simulink model "Noa_Nofusion_backup"  (R2020b)
settings: Solver=FixedStepDiscrete  StartTime=0.0  StopTime=Inf  FixedStep=0.02  RelTol=1e-3
PostLoadFcn:
  | if any(exist('dsrtsu_mdlpostloadfcn', 'file') ~= 0), dsrtsu_mdlpostloadfcn('Execute', bdroot); end
InitFcn:
  | , if any(exist('rtifpga_mdlclblib', 'file') ~= 0), rtifpga_mdlclblib('Init', bdroot); end,
  | , if any(exist('dsmpb_private', 'file') ~= 0), dsmpb_private('dsmpb_mdlclblib', 'Init', bdroot); end,
undefined symbols (not defined in the file): ACC_TimeGap_DecSetSwt, ACC_TimeGap_IncSetSwt, AccelPedalPosn, AccelPedalPosnVldty, AccelPedlPosnDiagc, AccPedalOverride, ACU_ShiftInProgress, ADAS_Posn_CurLane, AESSwtReq, ALC_SwtReq, BrkPedalSts, CC_ACC_CANCEL_OFFSwt, CC_ACC_CRUISE_OFFSwt, CC_ACC_DecSetSpd_SetSwt, CC_ACC_IncSetSpd_ResuSwt, CC_ACCSwtErr, CharSpd_ms, CSA_NODE, CURRENT_GEAR, CurrentGearValid, DiscIntNeverNeededParam, DrvDoorSts, DrvSBR, DrvTrqReqOvld, ECMACCInterface, ECMRespACC, ELKSwtReq, EngLimpHomeSts, EngSpd, EngState, EngState_PHEV, EngTrqMaxActSpd, EngTrqMinAct, EPS_DrvInpTrqVal_HighReslolution, EPS_FailSts, EPS_LKATorqOvrlDlvd, EPS_LKATorqOvrlDlvdVld, EPS_LKATrqOvlDlvdSts, EPS_SteerMod, EPS_TrqSnsrSts, EQ4_APPINFO, EQ4_LA_ELEM, EQ4_LA_HDR, EQ4_LAP_ELEM, EQ4_LAP_HDR, EQ4_LH_ELEM, EQ4_LH_HDR, EQ4_LRE_ELEM, EQ4_LRE_HDR, ESS_PedSwtReq, ESS_VehSwtReq, FFogLmpSts_F_Pbox, FLWheelDriveDirection, FLWheelSpd, FrntWiprSwtSts, FrntWshrSwtSts, FRWheelDriveDirection, FRWheelSpd, HazardLmpSwtSts, HCU_AccelPedalPosn_Diag ... (+152)
libraries: simulink x117, dsmpblib x30
(part 1 of 11)
PreSaveFcn:
  | , if any(exist('dsmpb_private', 'file') ~= 0), dsmpb_private('dsmpb_mdlclblib', 'PreSave', bdroot); end,
CloseFcn:
  | , if any(exist('dsmpb_private', 'file') ~= 0), dsmpb_private('dsmpb_mdlclblib', 'Close', bdroot); end,
settings Model: DataDictionary=HWA_DDs.sldd  RTICANMMDATA=struct('GeneralSetupData',struct('modelroot','D:\ADAS_Store\Project\adas_project','generalsettings',struct('filesettings',struct('destfolder',struct('Name','RTICANMM_FILES','Check',1),'buildfolder',struct('Name','.','Check',1),'AbsDestfolder',struct('Name','D:\ADAS_Store\Project\adas_project\RTICANMM_FILES'),'AbsBuildfolder',struct('Name','D:\ADAS_Store\Project\adas_project'))),'options',struct('addpaths',1,'rmpaths',1,'addtrcexclusion',false,'cannavigator',struct('checkmonitoring',0),'show_usrtrc',0,'use_usrtrc',0),'advanced',struct('options',ones(1,100)),'MPSetup',{{}},'RTI',struct('Type','DSRT','Ver','4.4','Date','02-Nov-2020'),'modelname','Noa_Nofusion','block','Noa_Nofusion'))  DSRTSU_INTERNAL_RTIFPGA=170  DSMPB_ID_DATA={'105434',struct('BlockId','e4345bf9-5197-4b1e-bd44-61eb3726c26b','SignalIds',{{'26e03e37-8c74-4456-a1ca-96577a784511','08c7dde7-a79a-486f-a58d-e9b634b8613f','1f5a9323-8244-4deb-bd12-eda6c6bbb4b7','bc7a83a0-3632-4f82-8cb2-387644efddca','463d03f2-aaf4-4ca5-834a-63a22e0dbd24','ff01abf3-987a-416d-8eb9-6d8f794c440d','a2437182-dc0c-46c3-ac4d-08683593369c','67741761-aed5-4514-b3bb-eb9079150845','4cc3f4fa-5aab-4adc-a725-9d1cb733df4e','fdc02adf-bcbe-4b15-b2ae-adf627f92255','a032f0fc-e186-436f-afc3-d181db7ca0f9','1cb07c07-79d8-437d-98ef-a715fe9ea012','b05a5e47-f50f-478a-a637-5469c5388606','f41b7890-420b-4a6b-8009-0b5652f97978','d622c0c0-f466-4673-93ce-b079da25035e','71aba0d3-083a-41fc-8fbc-153153d0300d','adb1eff1-8bdf-4208-b3d8-aca34dde9050','a3da7591-6b53-4fcf-b698-0e5273c81e81','a998d2a0-6de8-4bd6-b5ac-dc2d5f8f6b74','5e2ab582-2ba3-4786-882d-7e45b79ee759','0c4ff3f6-444f-4552-8419-c424fcf95c3f','d1700e2b-2e44-4df0-90ee-8a8e8a240ee1','4011d0ea-7b24-40b1-b899-1ec42639ad6f','c062954e-3331-410a-8824-613eb22a1fc5','16bc174b-a18e-43b6-985b-a64a73e0a52f','cfaca706-1dd7-407d-a107-3e9967b0bc1a','a67fec9e-f77d-4ccf-86bb-46fdce40b352','150cab41-1ab5-4854-ac2c-feddb3f5cac9','58e8d9c3-1336-475b-a3f9-01b1e0314959','42e83e1a-7335-4d70-b47f-232895adc5a7','e777976c-f6c2-4f04-a8b7-d94d8ccf44be','91bdfc1f-659c-4474-96fa-ea1cd21ec91f','20a78a99-30de-4c30-936b-ec269208d6d7','8b4dfdb2-a3a4-415e-85d2-0017a012fe9c','bfe8ea3b-4428-481b-a2cf-ef431c2d4e88','a4dae870-9959-4a91-8cf5-9cb1a03dd0d0','bd415c22-eb37-430d-9fba-56a2024eab30','32c5bc48-1ef1-4e48-92fe-e0b8bf641969','b8824d59-4ff1-44f9-9d43-98ccd1ef7818','2b530dc6-df14-4df3-a10d-b6a7a38ee3a9','47fc8431-8e5b-40fe-9bef-bd4f615a5465','85a00529-8abf-480a-b50f-da5245136546','75671914-23b0-4c0a-acae-2b7d58b763e3','69d46c2d-3b92-4b7a-8592-6c17caf294ed','18268954-c92f-4566-9cfe-583b74be0081','2fbcbfd7-1e0f-462c-b4b5-155ea0e0a8e3','851a228b-4320-48ca-8076-5eaf54d60810','99d04a46-e5a2-472b-a0f2-fbb65c8254da','e47a005c-a981-49a8-95c2-c7622c1b877c','b894dada-0a4e-47c5-adc8-0014d2607e23','0ac0dd78-1a61-4124-a84e-c4d508ff7f6c','dfe863a0-dbf9-4271-9fdd-b9d8c3f7cc2c','3669fba7-b792-4083-b91c-6483b65952fa'}}),'105435',struct('BlockId','d40121bf-53fc-4e4c-bf6b-9841f4415676','SignalIds',{{'cc5a11f6-e480-49b4-bcb9-da409be93ad0','e485a1c5-525b-420d-b245-0bdec7efe4d1','7063e335-e5a3-4215-a027-5b046a440513','370c96c2-c68f-4ad4-b008-588ba83deb3f','29c9a21f-53c2-4740-9418-e0028da600c3','d2ec761d-b188-4679-8bab-e24c9a56caed','fb0e0b0d-7187-4054-93dc-12a477d09059','0587543f-c20a-4b2c-a9d7-421455e1177c','c6236804-cf03-4372-979f-22949d9ffe47','dde724cd-4d84-43d6-9098-33f65af196ff','456acbbc-8be7-49b5-a0d4-6e3481273074','0fbd5400-87a8-4635-a5b6-02b9f8aa8a25','70bf8bc3-6666-425f-b514-d1e4a0a78933','6f4a0559-72ca-4952-81c7-e8c921498f82','ba6e8235-f42a-4def-b53d-6a69067deba9','3d993282-3ed7-4dce-a9ee-645c134cd44b','0cc06f80-c240-43a4-9b8f-4f6b9595cd8a','053b5169-944f-400b-bfa1-e4821136ec08','57d9f0be-2eb9-404e-becf-fcabc8470df5','b6e2025d-94a1-4f04-bfad-ebc0c3406e95','d9141aee-70c6-4284-a507-75d7f7a00e1e','6081e494-0e08-4c0c-ab2a-c6f970f11c8d','9fb5f869-4a24-4422-be73-f89fea30026b','a31ae767-f7c2-4d08-b138-f5b138cd782c','8978b272-f1d1-4dda-9a18-2e5bf203213e','fcb4403e-c5c0-4e63-a493-c28f06f4e989','e95a9918-a651-41d3-ae0a-66028e446d9c','83432099-6253-4fca-888f-af4b2b218d19','42653c93-2326-41ae-baca-2973fac6a4de','8836ad72-f3ce-4aae-b8a2-47c801e52c02','b0c13cb1-1574-4c16-b62e-ae7ad4d8b61f','283ef39f-4105-462c-ab0a-cf33dde3f661','3b3621be-a1a5-446e-a438-ee9142b86be2','43a4c43b-4ff0-45de-8a39-183cfd89222b','f08aa7ec-d521-4475-a3ac-08ba9d0ef18c','b2db309d-0a89-48d7-8b02-3a67f6913b10','2755c593-1eee-4c99-b46a-f03229636a7f','e2fd6a35-f7f1-4726-95a6-4e08663ad70a','abca7ea8-e11e-4d27-af8b-de618eedc876','b658c1af-14c2-430b-a331-ada145c0fea0','f98fe55d-f2a9-4261-90b9-8c4000dd9d04','688c6ece-80a2-46b2-af42-176bf1f9fd39','e9d10bd0-a7c8-403c-8590-31b64efec433','304f842a-dd0a-46f4-9fe1-0b3ef7066bf8','7a2840a9-195b-4485-bc10-ebd18e7a7110','6d0cfa48-0ecb-4659-a5ec-3cf69aa05638','00a37eaf-aba1-44b0-861e-c63e2cf71b26','f01dd479-691e-4b24-b10f-fb2a411ef3f9','bd845b67-c975-41c8-99fa-8d1e7106f6bc','4f7fdd21-b181-405f-9b00-d96648cb766b','f3389090-f0b9-457c-85ae-bcafb5f9c756','4657600f-e2ac-49c3-8fcf-c6d5ad3031eb','1a617fb4-0046-4c94-8581-01a2871ceae9','010eda22-fdee-4a99-b239-11724803971c','a9e798ca-198f-4a95-aa52-b8bf9c198389','f780cb99-b180-495d-b16b-9a32fb4fc008','946e88ec-8a2f-445c-887d-8b232953bb76','0cf59188-d479-4f11-b384-9398ad11b0b9','b429280c-67f5-4e1b-9e7e-07e7eafab7b3','c68f2587-46cf-4460-91be-325a9f6f0058','31916026-ab7c-4d26-b8d9-7c0947af4bb6','4056ca2d-ee20-4a0e-b887-5f2d42dcd476','0722f49f-64d1-446e-bcc5-e32cefc2cd07','9aa8ee7a-4d05-4864-bf05-1bde538fb5ef','91f59306-c587-4cfa-8cca-f2fa2bb27640','3ce34415-7470-4bbf-b6a0-34b9c9680686','2521a64c-fa73-4f46-8f58-43774ca93d19','22f357ae-cedf-4c71-a114-455f7eeeb852','f33afee2-1018-43a1-b2f2-b8249068a706','a3099f95-10d5-484f-9bcc-6a12ed409148','1c44e4b8-1a98-47ad-9d1c-ea3a539f74b4','cbbdc108-b603-452b-a824-5e42f89503e4','fff7e395-1071-48e3-909e-1e745a3936a4','a01a96d1-a628-4ae1-bc97-285a27885103','98d1c28e-f030-4320-a1d9-6263669e6f95','d3664eaa-a3c1-4179-98f6-7c6d4c30bddd','813f9209-a7ab-41be-85e3-3427ba85c434','18fe41b5-a649-45f3-bbfc-b0dbc7cb99ae','72475f52-be41-464a-8f0e-e9a62708a4e8','dad4bb40-ec9c-4aaf-9fc2-0712ec0f2241','4ab7dcd5-e52e-4fcb-ac29-82510b47df2f','7a00036e-29f5-4968-8d52-2a0ca2bfb714','4a83fb4c-b02f-4893-a8ea-dc9fd0347245','1294e5c8-6cb6-4f97-af30-ed027a407515','c1586ad9-805f-4123-af29-7bd37ac08373','fd82f8eb-65d1-4726-94d6-6ed5227b2f44','71f76165-f05e-444f-b18f-bd431ae3420a','9ca8daaa-938c-4c2c-b40f-9abb9fa373dc','a275610e-c197-4c68-93df-f8647aab9abe','4e816bd2-5b5b-4838-8c15-47e708c09655','107a9ec9-74cc-42d8-9479-17c41f92d23a','3f69883d-5772-4566-8b65-fe213494fc07','1acadf61-6fdd-4c01-b3d0-7293d5cf0b9d','fb5d8406-dead-4a01-914e-d88103fdc350','5b74708a-44f5-4ce1-bf13-9f0606d646a8','849bf2a4-7bc4-4e70-8423-14ca390664cd','a62a9267-333d-4d26-851d-bc457f3b81f8','1e129e98-37c9-4fc9-818c-296032360fc6','a4650b49-c80e-4b85-9076-c990629bae0d','c0ee05c1-f0cb-4541-aaf7-6d6b08f9a5cd','e2d169c4-0d8b-4400-a269-692e3f91bbe6','492a74b3-4d11-4662-8c3b-fde7cb230339','819494d0-34e1-4282-a222-1b52ba27ccab','5a638eb9-ccad-4d4a-9718-d37c62ee852b','c803a847-ecfa-4cce-960c-e106f0c4ea6f','e886af01-08d7-4704-a3ee-2d930691e91b','96070339-ef94-4b80-bb03-79310102b68a','b439ed2b-cdd1-4b08-990d-2a205f128d33','032805cc-419f-403c-9f6a-0eca3a183b61','88916648-e457-4bfb-9eef-162e217cdd8d','0c495062-db58-4a97-9a48-9d285bff8853','a627fe6a-96e3-480d-a583-a27d3bea5d25','799f7d78-721d-4d18-9b5b-df25b89a1a24','0365b900-2f19-45b4-8da9-34546021be40','0fff78c4-c430-446f-9f7e-7cf1c2560c13','bb3dcfc4-42bd-4e8e-9b87-b5baa2fa9966','f58a7d4f-359d-4f5a-a673-ecae1cec1cff','29bfd316-2c17-4da6-ac7c-92a41147bdbd','10fce9c2-b244-4020-bbae-d37dc28ebbc1','02e3f3c5-b52c-40f5-bf8b-7c169b6a050b','d1869188-5151-488a-974b-611ef2b3e735','3feb2bce-f837-4d53-afcb-2f51abb1249b','17ce8e05-201a-4ce1-90ef-a5d5fde36f30','cd40ee62-3fd3-4019-9f81-335d24b7e533','77bdded1-20d9-44f7-bebc-305e6f8a7542','7fb625b1-1694-40d9-8650-06db9adf04b9','0e5ce812-dc7b-4bcd-b991-c5485d68b836','fee2eb9c-0478-4758-b416-366bfd0a0b08','36b53c99-ed23-40ea-b736-d6080d358e52','7a9ac993-3f27-46ec-a0be-48db83299b68','720de45d-04c1-463b-9803-ef9b2b0640e6','48dd3c23-1521-4de4-8c14-bbfe09d8cdd3','0cf887f5-6df1-4e9b-89ca-8de50e244c96','d3e92529-0445-49a6-ae88-b8db65620ada','00961a9b-8e43-41d7-9361-0f7c9a191df1','176a2a26-953b-451b-bee7-639fa5dcf115','05743b62-48ad-4976-855d-4efd760ab5ae','5c8a3068-7b46-4863-96ad-cb43b0bebbf8','7e50c02a-d315-4f98-9ab4-c963b22f5fd1','decd5ca8-ac57-4887-88b5-f572b41815e6','7df3046e-b8b8-48de-bf08-08b163efbe98','068e11f8-fc7c-478e-a264-2eba7fdaf707','75e971b6-9816-4b6d-894c-7f0a5e23aad8','1245d556-b9a4-4269-8015-ee1cf4c77d66','e7a9388a-c9d2-45d1-b0c1-14f92e703417','e3451999-4f34-4207-a06a-a1a02f4ebc46','095f9967-1705-4584-a3c0-0a7a58bb2f86','a03cfd89-db34-40c1-9760-adbbbd92ecf4','2f200d12-fadd-4c60-b392-739715aba906','dab68d27-ce17-4104-94fb-d9520fd1074c','19930cd6-7971-4ea0-b243-faaedad380b0','81ee13d2-2426-454b-896a-4e968cc2b063','2182b590-601e-4655-89eb-6887a470e591','1cbdb8e1-bb61-4c18-a563-629debd208b5','94606876-5750-4d63-9bf3-4013ab9917c7','3146120c-38a4-4420-939c-eda38ea68cb3','cdb35835-5fbf-4349-a86b-fb87a21169b8','d21c81c0-6dba-44be-b882-848afe41626b','1201d19a-6fe5-41bd-ae3a-bd6a13dff8b8','91a5b005-6117-4516-a073-8851c35bf8a8','06b71312-9340-475e-b4be-cd3240c14140','23eb5363-a588-4710-961d-f99ccdee6ff8','a9d3dd51-03fa-4728-ae9b-f934500f1552','7be770a8-e416-43fc-a2aa-3a7b7d47063f','b1cd6e8c-2dc7-441e-8774-2b064ee9434b','77f2dd4e-5295-4873-839c-2804f01636cc','ccb8cb5c-6d49-4f47-9128-08c71a8596c2','68b38d10-57c2-46cd-a9a3-39ab701353d7','6d2417b2-923b-4307-8e62-1a997f2a7e41','057f6026-574a-4c10-b798-8674bc70fe4a','4ad31521-ed04-4046-afa9-acec64e978f6','53b9bb73-2211-4cd3-9be8-cc07ee60870f','fb200ae3-4897-4a2e-aa8f-753c4cb12daf','f1dd6b03-29f1-4510-9072-d50a6fa7b5cc','b4da77c0-2abc-4e81-9be0-4fa0d3784d94','ece98af3-fed9-4289-8066-50dff056db58','021a28ab-d2b0-4e56-906a-085143f1e294','9ad79b1c-39a9-41eb-926a-7326bbcf277b','6607879f-b8a8-470e-baed-66e05d35583a','fa2f7a6f-8388-4a48-ad80-d1f0da9fad28','d494d8ac-ce0c-4623-bb94-131d0977ba58','0cccf5e1-0fdc-4153-9508-5cf92d457e81','7407a7e1-6edd-4d87-b55c-fcdd84c2983f','9a18cd5b-06a3-4c13-9bcf-7adb69bb1915','453e0b8f-8cc9-4c76-9632-9981e365a1fe','a1003730-fcc8-4975-85c0-d51f67bec0e9','d1e041e3-d630-4ed2-a4a1-3340570a9861','24f6b2e2-26d0-40b7-91d3-4d06786d847c','44224ffc-9120-4fa4-823b-43d88ecfae98','ed8d8980-8de8-47c8-8352-9a2594ec7e8d','4594a42e-3277-4356-960d-db7f54018581','b7933dfc-e99b-4671-ac5b-0b539745cf2e','debde9d5-90eb-48ab-b125-b2c5ad0b1089','b175ca9d-34d9-40b6-8ff5-919b9d14b24d','5177fe90-62fd-4f07-9408-1db74678403b','439b298e-d093-4fc9-bc29-09baf018ca0a','fec7866a-292c-4ddb-8b2e-f6973b69ef06','a11ede85-44f0-4b05-85ec-a5bd55f71b4f','a0cc3722-caa3-40e0-a9fb-a0bf80e1730e','63ffd194-2be4-4603-904d-59907a931c27','d969c761-cb58-4b59-b72d-b3777adbeb2e','fd61477a-d646-4fa6-aa14-daa7a0500d24','e597bce3-f71b-4756-9897-14f096504c8b','c8c59d5b-acf9-4b59-b898-f2cf904d292e','0161e9c2-c134-4633-8f84-d49d04144a87','8b756ca8-0e95-427b-8560-8d1f79dc86da','9fcac863-048e-40ae-9155-08ed5010dc46','be979dbb-77e6-409c-8d46-a282d6d7b717','9e1fe4da-8bf4-415b-bf54-a00fc9538685','6ed6f9c2-07e6-42c9-9d33-83aecc381688','17e8478b-6bb3-4189-9dd7-157df52c13c6','f1bdca73-12af-435d-b22d-32002e65f1ee','929a8c7c-97c0-44c7-8c79-fd6a80dca632','413238d4-e9da-4389-8fa2-056224cdc256','56cabf32-638a-46a9-abe3-0f9647e0cd12','3ce98a47-237f-42c0-ade4-ef06ae0e8951','eebaa124-7f65-4430-9871-33a15f887caa','d4e60423-8c8f-45b6-b121-b99db76df8fb','cc5a559f-a448-4899-906f-5dc9e1af9340','e974851a-54fb-475f-ad1c-f92776865502','ca0cf790-84fd-46f7-a553-c999687b713a','8ca16ee8-27ae-46d4-8d1b-6484f0ba2e1c','759c7fa4-ecac-423f-8cc7-22d8663b1b7d','a32945fc-842a-404d-b759-2c4082d0afb1','a3e8dd22-699f-447d-8e26-c3e63e8cdf8d','c7e4f5ce-5fc0-4b2d-8595-25b0d014f116','2afbdbf5-e43f-49a0-92c2-dbf86f141ee2','a67f7783-5f44-41b0-b0e5-610b7cd4cf93','28fa3106-f248-4371-864f-c995c3c6a1d8','c92b734f-8e2d-4b7e-9242-c73c51499704','41b74adc-ad96-4fa8-a326-67da154d2e5a','9c6b6b81-d000-40da-a81f-97b7769edeb7','3fcb895b-97d5-422c-8812-44e5092a1c13','425b0fc0-c480-477f-8574-0f601cf6a832','ac0d790f-a75e-4b8c-8140-f1a1077511fb','907c9527-8a89-4c72-9ec5-032b21f4476e','01f35774-1138-4815-9226-b549d6d07300','9c2c0849-8eb5-489f-9256-4c61f1511d6c','691b024e-ea18-47b8-8c91-4d9a84de3391','8ce8ee90-d8ac-4999-be4a-3cc9b1a1ddd5','330b6441-7005-41d8-8d7e-c2fe0fa98f1e','097751a8-dab4-48de-be29-ce5c72bfa38f','ea9e5656-c12c-4b65-b5b0-27911e1a9074','d894742d-141c-4ca1-a31d-14590af5cb88','18db3a2f-1f99-45ff-a28c-9d4de5ca09f2','bd93bda1-440c-42c1-a94b-31318096355d','c9010752-1ccc-4f48-9d88-00800dca04af','3dbf7699-72c3-4cd8-a1ed-344c2b193fab','6e11cc67-229d-49fe-9524-842e8beb6dbd','5c6911d4-ec52-457f-abc4-7531c8e96b32','3642b32f-b4ad-4eda-87e5-e57e269a0737','3ce9a289-c5d9-4dc9-a836-09cb77dba024','6b1c0f1c-5802-4a48-928a-7d14e45f2140','21de2f49-14de-4bcd-bfd3-ac7f7ebcc380','3585a489-3f47-4b9b-99f8-630657ca6b61','d2933102-4f42-4f86-bd5e-5f2f55fca8a9','c441195f-73a4-4dde-bfdb-1e99f2d402de','2bd35363-f924-48df-9bf7-0ff957eaa548','8fdd4ce3-583b-4977-bfd4-267de9e56221','da41d479-773c-4ae6-b31c-6f2c310b8697','5197f87c-2bad-4e3e-b8eb-1dee0cc507a1','0b6746dd-4b7d-4483-b390-2596ea9c94f6','d3aaca7a-e726-45c6-a876-1d36405328e8','e4c351a4-0d06-418c-b290-86601264d4e9','98a41ba7-8f43-4ee2-b203-f62db5551338','319d5c62-7a79-4fd4-8ace-256e219e7927','a704a474-bc59-4be4-9c29-cb9a85f8ed60','0b2a3c92-dc27-4033-9d0f-76ea27442d02','437b8219-2177-46a7-8e27-d74badf66ad7','bdfda334-42ae-4382-a6d1-596cda2fae0f','3ce29b3e-42e1-40a8-a4a5-c1706b66ef27','c9c7185d-6b37-4c0a-8b35-64238a1ec5cd','76a3b79d-a942-4f96-8d54-397cb6d54134','69332480-af1c-4431-8c89-956bc5b9ada2','b90b99c2-80b5-41f4-b872-e8d40f6b986f','11904823-be19-4a56-b728-0959cc99c2dd','007e0102-eb7a-460e-bd55-efc54a9d09c9','2dff0e5b-5a66-4099-a59f-03486706e809','ab438635-fcd0-49c1-b5d7-3a38a6dd5d6c','a8ce4e02-4111-4410-bb37-aeb5015d0f28','4612e75f-7972-4b2a-b0d7-cc8e529f0a42','0946edce-7d00-4b41-9bc2-d0551a007d3b','838dbe22-0353-4e26-a393-dea5335713dc','eddf385a-eb65-4c84-8f9f-cfc6e10ae678','83670045-0068-4c9d-9d44-ca98496249c4','6ad6d159-db55-406e-b158-d7decc68f78d','22db6a37-3350-4ca4-a97b-07980acf5a21','512fea98-8afc-49e2-a79d-9818b29f3894','692e8e3f-1d4a-4455-a7c7-e545a1ba0b9a','251c595e-841d-428b-ba31-7c6b9e852587','764d5c32-5c5e-4761-9071-007a4bc162d6','1f53d17f-2a1c-4bee-8a7d-dc4d7147df35','e51b0e47-7399-47cd-b026-f67ad625f364','2861a8b7-810c-4ce0-a0c0-b0502751c142','1c517d95-89a7-4442-9e57-b93e98d12f2c','8a9ac90b-68ea-474f-aee3-1e5008fd098d','d0c1cfbf-c955-475e-bed2-714d1c907249','74d6c0be-dcbb-4737-a584-266dd9978f33','b654b6a2-8011-4d6c-8572-18d135e251ed','91b173c3-804f-4276-9f17-2d6da234f79e','69a1db0f-61e5-461f-bba8-b382b8817f9d','c451186f-65aa-46d6-9d99-cec024e2d63d','79c91a5e-f416-40d0-976b-045ec1d133d9','c2a92a7d-2bd8-4d7d-addc-c31bbe7b2e06','add2c099-0616-4f5e-a06e-a2a69bd83097','a85fa2d7-93f4-4009-901e-c7991975856a','9b79f2a7-b3dd-46bc-b8c5-92d7ffe34ab8','e61b549a-71d7-4ce5-b867-e409b4815d6a','6e0eb462-856a-420e-806e-2aefdaa6f9e9','59708c7f-a4f8-439d-bbd5-ef006d9d94e5','53a689a5-895b-4661-a768-18b97131f9b5','d63e55a5-23fa-4d36-848f-48eb2a0b39ef','01c1f276-f558-49cc-8256-1ae84a7c9a8f','fb911f03-0812-43ff-be03-aef72409e834','53ca8056-b924-4d6c-9003-fd141a5a0e09','f502775a-ea5f-4fc8-8f49-0d44588d6923','fd9a4963-42bf-454b-9105-f84f7d212dbf','8d2ad19f-788c-4d41-86a3-6f5092c3659a','c0569295-9bbc-41d6-9c4d-9217cc984067','08af115d-a552-4fc9-a13e-9bbb52271bbc','d5b4cbab-f87c-47a9-91f6-fea75233e2d1','17487a72-6383-4c65-8972-21fa963fbec0','10d55baa-318c-42d3-a564-e728fe9d2880','ed40f1ae-203a-4951-a78c-f63f8a19583b','8a0734ac-6aaf-4db4-9ab3-f1d7de829468','9be2a3ee-f28d-470e-9b68-7e167ab84867','c4ffb54d-ed0f-457f-851c-5f221df9afce','3486935b-dd1c-489b-bbd3-73e6da203050','405ea1cd-827d-4205-9f8b-6d069b3358ef','65b16e84-ab72-4179-aea2-fbfb6032235d','77256c6e-1bae-412b-8946-ade2dfcd8b2b','a8569a15-8d34-4499-a902-3b93742385d6','29f4f5f1-a2f0-4d17-a8d2-e5bd679a6191','32be050f-77e3-418b-8fc0-01d52c0f81b1','5299eb59-fdbd-40fb-a2de-98847db328fd','c2270d11-788e-4144-9bfe-f73fc87d227c','f4e19d23-2bd5-45f8-a648-acae3bbe24a8','ce4d68ff-941f-4558-9f31-d5b994b2288c','32445c74-1dc3-44dc-80ff-d2d906b6c70b','3e688b65-7195-46bc-af07-3a64420f53b6','e63a5e33-f993-4f75-82f4-28d25c86114b','a10fa038-6d5a-4d31-a99e-1ababa1005ec','b4a17c3f-7bec-4608-93f6-1a3701a46531','afca4047-6d67-42e4-a93d-21200c4aa8dc','14830bc3-064a-4486-b298-24319e1b19e4','7227227c-9520-4bb3-ac59-8e658092cb02','9b8b4492-a383-43ed-b6e9-5de3f8b2d5e0','cf459a79-3a7d-4d6e-a941-a4e0299de77e','5f828eec-cf46-46a6-9017-894a0d3527a0','db4f20b4-b889-454d-a614-d932461c028b','e7defd96-dc06-4b27-b5c8-0cca9e849e3f','5c1cacc8-6dc4-4385-939f-f931d9898e3b','f2f4044e-2c02-422e-a838-b2c8cb3726e1','93e34572-36f4-418e-8e83-15f4a80aff5d','2300ce0d-9c26-4d74-a513-69e4f5a4cd51','e13b9b7d-ff74-4822-8ac5-33be9ab3de9b','30c78f0a-e43b-4ca4-a84d-6db014e323ae','872e4fe2-02f8-40bd-bd6b-e2ac1f3bf7aa','e8115592-43a3-46d2-b96e-27f73a6523bf','43175569-a76a-4ac4-a1cd-f6b9a9e75f9e','42b25d4f-daa9-4294-a50b-017c03fda841','8ed3fbe7-accd-404d-8895-c45f61cd0cec','f68c054c-bb02-42c8-a359-37c399b89720','87971450-497c-412c-bf6f-8b77d211ec78','87db29d9-3059-41f1-917b-22bf2a621b77','3c6509ea-4a7f-4b60-9eb8-89f60a25992b','94f6b9b8-e704-4ddc-a645-cb1ae885c6ef','0948a254-3f43-4540-8864-8dd051921852','f9fd1072-82c8-4ba9-a8e9-745ab72c9d76','ed2d49be-d164-48bd-84f7-69a0a497bce8','545e9a80-fa65-4761-beeb-1097ab7b8a0e','bc2f1593-2577-4309-b83e-d05fee864886','2fc0fbbd-b198-43f4-9475-a901d5a10df6','9448c0e2-d8b4-4b68-97ba-7566a4a369b5','2474c5c6-41bc-41d2-aad8-465a46f2299c','524230cd-ca9f-4540-a678-50e3a691675a','35027490-03c2-4e93-9285-d408e3c85e64','5025e79e-722c-4608-b43d-2901a71948d0','b0480f38-c56a-4d59-ac9f-ee8a3a1c57c0','1f90e26d-0793-4665-a0de-7a98851a40b7','3a1ed6d3-3604-4d4a-9fc8-f094d7b31959','75b3eeb1-22b6-4b60-b443-5fe2744cd2df','44c2b35c-5090-48f9-bcaa-8050a1aa8fce','2b74c30b-cae2-4bcb-9a6a-98002332f100','547621c3-903e-48fd-a997-48378e062f62','fa9d664d-76fc-4f25-9f93-7dbf800054b0','93723c2f-03eb-4897-a44c-6d71daaf449d','ee3dc453-bece-4de9-b121-84375ee9e7da','fd4d0393-b60d-442f-bbe2-0f7f41acbc47','276fdf0e-63b2-4701-87b9-5ac3544636da','0c15af05-1b72-45e1-bfa5-9f7fe0e5fbd2','b9b2465d-5d27-4f91-913a-bee1615fd701','8df75123-e18f-480f-9d47-c0cb24e5dee7','77900ef1-cac5-4a18-96ec-1e3969270f79','024ddc86-7b33-4e29-8e87-0331e33b85b9','eb91361b-cc72-4174-95d9-9350d6ba38bb','1aecc688-47a9-4060-b8d2-3c94e7dbf89b','38ea6185-827f-4fa3-b4c7-83b5994143c2','f0517fc1-3e6c-4f3a-815c-dc1aa8a54192','d6c1d36c-d6e8-4461-9d0e-865617157fc6','9002abc6-6fca-4f66-94a4-ecabafa6ad9b','a1b25a5d-d9e8-40ed-8aa2-53d788e19b80','640fb393-c1b7-41f4-865d-09736c3d80ec','2fe3441a-504b-4e78-9135-3c2fda2e2fd5','4a6cd03b-2dd2-40fe-9040-0f0de504e462','3129f584-06a9-491b-9699-308a3f45a965','872ad8ed-c974-4495-ac7e-2a5b2ba741d9','20d2934c-1584-4be4-9879-ffb0fbe83803','e605361b-6cc4-4f26-b248-1db43a5454aa','fef12649-2b55-476d-8333-d82f5b554505','9cd47144-1de7-4899-a9e9-97d887f8d469','1313e814-b848-4453-a121-d9f1a42e2af0','0857829a-9dee-4edf-96c2-6b6bb5e76e34','8b45f3ee-ca72-4f72-8edc-f82059d0336c','9282acc7-127b-493c-98bb-8d88a1013977','945d9a30-6007-43d8-8e08-e078ab5d64de','a3fa0d28-3aff-4251-ac7d-7c64d54c7559','6c2ebdd8-afeb-4ea2-aa66-f7da39f68241','872b1e63-7e3b-41af-a38a-3982289009bc','3b7278aa-5f7b-44c5-90df-cd506fa3f5fc','6e30a5ac-5d6b-42ae-87b0-afd320eeaeab','0a6da5ec-bd82-46a3-9eda-f18aebda6601','78517c35-3059-4ba9-971a-45ff1196bccb','f79b8480-ffc7-4d29-b810-bcec72590bdf','093d2339-c1b2-4c9e-b437-c400b15b4f4d','eebb9dfb-1c5e-49fa-896b-e5fba41c1b70','1fa49630-a0be-4d70-9bd4-d900160c129b','4df3d1eb-f3f3-4780-af48-82697afcfa11','177dcbd7-e619-4a30-9b13-afd4e8f4c2fa','5e930fd7-66a6-427e-91c8-105a61db1d96','645914d5-a509-4680-81ab-634d41dde3c6','a2e12e22-9ba2-40f4-a1f7-4665d552aba3','debf0d17-6936-48bd-9d3f-d919662e03ec','8c5a8513-e35a-49cc-9947-5a1ff1e951e9','1c774eaa-e026-492d-a7e1-166124c32074','f5ca4b0d-deb3-41cc-accb-9a1ee16adc68','c96534b0-3f4a-44cc-bae1-4a1e802d61bb','038c2574-5fac-4a3d-8ba3-010f8d57dd9c','e91099a2-4c9b-48a5-8441-7df00938d62f','328eaf6e-c2ad-4ce7-b942-5ee57fc74870','f0947079-c6b9-4f20-aa56-bf3017b22ab4','b7e450fd-76ee-4981-a166-6259c51a50b4','ff84976c-67b2-4e04-9479-0083e5aafcc6','a8b0654d-e895-43fc-a680-2d8c731d149e','181a7022-ad56-43df-9b78-b64aa88713be','fc1bdf5a-b163-4486-9b91-03b0ab9c4023','ac8d2dd7-6153-4b07-87f6-4c3afed3e8e5','aa078f9b-9919-40e0-916e-c537e33a147b','b1873af7-21b3-4d95-b938-327be1c75b3b','ce70938a-10a0-41ad-943e-05e03baff434','f98eaa4c-5183-43f0-b63c-14b71790f611','b28686c5-02f6-454d-b057-1d675bdb81dc','e501155d-e3db-4bdb-95fd-d9622615055f','997faa46-b2de-4896-8e20-c2d4b8c1359c','fa78a12b-5d1e-4dee-bb17-1834b3c8f455','f72b09e6-6ccf-4d0f-a41f-ed679523f25e','d0021c27-2b6b-4827-b51d-7dae07425cd3','0ca30b9a-ece4-4689-a30b-96b0d9ce0167','96cbe83f-e04a-49c0-bff2-9623662c59f8','7433a08b-ca56-4233-a44a-5fa434f0b0b6','cda9548b-ecad-400f-ad22-55d4d1a3034c','492e642e-f9a2-48ce-b4df-bedb1adba8f9','d0eed24d-8ae1-4b25-8b6c-dcd5cf2c5ada','a4b28015-5085-4a81-8cc7-6144387ae4df','c38c694e-03d4-41bd-a9bc-a768a6c88d12','6e4029f7-4175-4233-98dd-fb097fa48970','89aca7a1-29c5-4954-9aa0-a670cc06e716','31944a79-b71b-462b-a6a1-9700eaa7b622','b2edd40b-d14e-4ddc-9b97-fd5aba5bd231','6bac8ba3-2f15-4911-8c3d-ba8376aa477c','f637f810-4adf-411b-aac1-4200ea0fe85b','f7602eb6-4760-46ec-b2c2-317c91bcc786','9dbcd6b5-bdf9-4599-a1b6-2e160dfa39ce','d2d6003e-c548-4ca8-a3d3-dccf5b598c1c','41daca08-c47d-4b8d-b345-a256e3c9be05','1f0b2279-0d5e-4443-8e9a-bc2fb4132a04','ec850a1f-c1ef-4b95-be8c-0e656818072e','7c975cac-4371-44ea-8053-0fd7bbd0c0fe','c243ed10-3bcf-49a3-8d67-2c142b11082f','5c646964-a426-41a3-9ce9-c215cb224a48','2d2fbae8-b398-4b6b-abfb-92d613fe18c4','a1435485-97e9-4877-b32d-304fb55e593b','94e98a66-7a74-4ced-8799-14727150fceb','b28c0b82-b79d-4816-8282-c74a0faeb3ec','f88e3e0d-a5c5-499c-a41f-2d1f925246f2','153af746-85d0-482a-b09b-76e153e776ce','5b91d707-8005-4e2e-8c86-118f89bcd2cd','36a32770-064e-4ecf-b363-c380a63312e5','11e4ff97-3c1d-4677-b9f5-389b298367da','c8ca6a3b-6d79-45da-a732-19ebe7540d7a','2f3df6e4-689d-42df-9d33-abf61f398c17','aeac4155-96c1-42fb-bc91-dc2c71c84578','2f8672f1-293a-40fa-bc35-85313a8da8bb','22dae23c-75cc-4ecf-a50f-aac362affbc7','c61b4382-846b-4a4f-a77b-e32e101667d1','611c4c25-17ff-4a12-8ca5-5537c3f7172c','750fa776-02e6-43a3-9fc1-ad672310e662','ab405c98-81db-45e4-80f0-a92434826387','e614b9e2-9e69-48a3-922a-c5f7752510a7','fdfda15b-f0cd-4cbe-b404-792dc2b0bed3','98f0ebe3-81d2-4b78-9d87-74cf0084b6e9','2e44af90-6a82-44c6-aa8c-2bc22f022714','61fc0436-4c82-430a-9722-a740790c8c14','370892f2-7549-465d-998b-a2ce99efc57d','f1e6264e-da30-4cee-a00b-a5f83ac3e8e5','066d2082-dfc3-44ed-b147-fc69905c3c5f','532d65e0-6f07-4992-92df-b9a9a018e250','1d3c285d-4537-4ac5-a3e4-edbdc625ce6c','08111893-6837-40ed-8b40-f1ef204607d4','74c0ee99-93c3-48fa-919c-c3a9f11ba173','de9b029b-0dc5-4540-b986-f626842d6427','a8cdf389-57bd-49d2-a453-f9dc5d1e984a','dcad49b6-d164-4790-ab28-5cdbfa2bb824','4a544db2-2a77-4ff9-a04e-7108a1e0bee7','181caa71-36e7-49f3-bcb7-56d2cc5f1505','b61f2922-2c0f-4312-b4de-12f0c4c94267','488d3233-de64-4ced-92c0-f77b27a88278','b7a15496-bf48-4f94-b60d-d9beda9e5839','2bf98379-1a31-45b3-9a7e-b57fea12a2cd','c1fedad6-6467-4ffe-a048-214609bc09dc','82097f1a-66e7-4b40-b629-4c21dbeb3a8f','d4f185be-a131-408b-8361-9f9cff72d4cd','3110e54e-5590-4dea-83ac-73b3a08d0550','4890fde5-f133-4e4e-a86b-6e5b7d44a980','08f31489-3abe-4937-92ab-b313d1c8c012','c145d1cb-19fb-4ff0-a8e3-e01cc887bb19','9e22bb75-4dd1-455d-b275-77b1b32c4e6a','34864cab-f8f4-4255-a26a-ac1bb9d8945b','281987eb-75a2-414e-b987-1b9bfddecadf','182a94a1-b8d9-4d51-8323-75170b59bdb1','9bb3641f-7eaa-4291-88ff-e1e3387bd97a','a6c1bac4-6fa8-47cc-b077-c21d524b49ee','a7fbbc63-2495-49fb-b72f-95b96116a0bf','1224b643-5da6-42ae-bbc1-55fe86bd58c6','c47c2fa8-0fea-41f9-92d6-66869a1b68d0','7096924f-0dfd-43cd-811a-980c70179f14','82158df1-abba-45cc-b849-4b2a0579f252','f300e8f1-a702-44b8-9dee-2712171c3a4c','3203aaad-c207-4d6b-9bd1-5bc965399be9','58ff5499-9242-40b5-bdad-d0e3fc167ceb','d443acd8-a96c-4fb6-ac01-451f0684ac31','f679937c-2064-4dec-8be6-f76b0e38263e','fd084c7d-eb86-4368-8e97-e1c7add861d4','95323bef-95d2-4714-9850-37a27cec1544','b6d7a45e-92d1-40fd-99f6-765a36cbb47a','f57bb77f-370c-4610-8cb1-4ddf2d9b3f74','1e8d914c-245c-4031-a0c8-f41917af18dc','85eda06c-09a8-438c-84a4-adebf7f77bc9','7521dc8e-0f81-4410-8079-d12e65789e30','e5049629-49f9-42d1-9f17-438bbc9e756c','fd432edd-8ed8-45dd-8c0f-7ca243305c4c','3ee7e66c-50bb-4821-a59e-049d581d339f','7522269c-3161-41bf-86d0-d958e12ac46a','cb333743-0f34-4d2e-8ba0-9d785247386d','398c7213-7966-4355-9cc9-7df5df0a75cf','d6994e42-c094-4dbe-8462-0da62a6a2e14','ae025030-5835-479e-a891-de27c637d219','61c95da0-80a2-46bd-97e1-9e6ad24f03ee','f2a29bec-b092-4ee4-9fe6-fce02dce5ed4','e269417a-cb48-427b-832e-5a14eb272aa0','6959e6bb-5c9f-4b9b-bd79-e26a56b76732','7ac261e6-cb91-4dae-90ac-c3704f71ddd1','6dd6c97e-d3ba-4bcb-b804-a10871f2db2e','21e7cfda-c211-4274-88b8-f3f4cba0bd14','a6123d7e-4449-4f75-bf5e-d90c2380af46','a18abd56-433c-454b-90b4-c4778833004f','efd2caff-f245-4b85-9947-5cac4b28862f','91ab604c-c6bc-47f5-981b-c349fa72b926','7765fab9-c597-4b3f-8c58-0b616b9aca52','32eb21df-1468-4f8f-b80b-0132e79946c4','23461d37-abcb-4de2-93b6-2c5b9b0285c5','2f82fe29-cbeb-4541-889b-8ca434b5dcdc','3aa5c75c-7fb8-475d-9ad8-74a6ef58f588','15702135-bba1-410e-9bd8-8a29575c5c9c','35d807ff-7560-4d31-aaf3-ad2e714f519e','f48fcd4f-b01a-4034-bca8-7150444f550f','36733f44-25e4-4e8f-9e06-a4eb4e366c81','9eb18c40-97e9-4722-8ada-89233fc24c6e','944672f7-8fdf-4c70-a203-1adb1ce43a88','46b707f3-17e0-4422-bdd0-c1515277267a','238ce7a8-54b8-4006-be0f-3c4ba43785ff','b4d4ebce-d852-41fa-b6b4-2d67323f73ba','480a575a-bb13-409f-8c82-179fad07672f','19788773-3210-44b5-bd38-6bbec63a8a33','2e9dd13d-b0c8-4b4d-b372-2c82b162cb3f','e675fb90-8b87-4e7c-85cd-6f23e0c28968','d593f8d6-dec2-4410-9bda-9b883f31f0ca','301d845b-2e55-4696-a79f-a33255234f38','15f9d93e-2322-4578-b26b-89a96a6236ed','e9aa8cfc-a767-4491-899f-76f9d70f9d6d','f6b3c952-7eae-40af-b06e-142c6ce86f9f','e59c1f00-1b72-4967-9c9e-0acfcff55407','3e5f55da-2125-4567-a48f-328cef8365e1','9e510b27-5ca4-450c-8f27-456defee6958','e1a18f76-2953-40fc-a9b5-cdc760845927','c032c242-3216-416f-98aa-6193bbda84bf','a5351ad5-64be-40f8-9ec4-28c814d50f85','1ed74a08-4f3b-40c4-bd2c-10e1ee884d6a','4bb619bf-cfb1-43c1-b123-98b1567fdeb1','4b011f18-a11e-4ac7-a14e-a7dedc986832','85c53582-83bb-43b3-a48a-5a6f6c021d88','e0841b18-6478-4e07-9646-269550b47938','1781b9e6-7833-4278-8d2c-4f594bde1b7e','e26c4ef4-feeb-48f4-8d5e-a5d95fed394d','a7e745fc-201c-48dc-8366-3909a9a9eb49','9aa2ed7a-85a1-41fb-b08d-3d22bb9c6891','732df68d-ef7c-43f3-a519-47e39aeef174','4a802f6a-48d1-4588-8e29-15de3154ac7f','415ae86f-fd01-457b-b544-f58320e3a421','0b702c91-2691-476f-ba85-0df6697a3b9f','85fb984f-d707-409b-9dd3-da8ada7677e1','db233789-2c59-4059-8421-3de4411cd725','683b71f0-ed89-4b04-94f4-685c7232b641','3b617c2b-9363-4476-8422-b6db119c47ab','6c2cca8d-cba1-4c07-a771-ccff85f0cd1a','82da558a-bdb8-4443-a0ce-db194c746cab','ecaa521a-d476-4fda-ac91-3b624d601546','61409ef0-4ffb-48f8-acc6-e1b0c4e8edb4','457e0140-46e2-4fe5-92aa-108d14ea393c','862d9e50-d7b6-4c9d-8da3-f1d0e49b0e5e','4b3e35cc-b9f6-49eb-87ba-b427a0508b6b','d8fc8946-2534-4323-92c0-dae9cc9180b7','3f48a1f4-7063-4579-8cab-e13c56a88b91','50b43527-8148-48a2-8e3a-91546cd4bb1c','e3c0dd2e-1907-465e-97f3-5b59e5f4ff21','7ca38626-1325-4058-91b3-c34b2161fbf3','25f87f8f-3f4f-4634-8a55-332c91c9fb16','7316b1f7-651a-4676-badd-533b941736f2','7c848042-facc-4541-98e9-4e2b7d739da5','069971df-605b-49e7-b9a9-92ab901d7663','c2a809ae-780c-4219-8073-f231c4026a36','d3fe212f-d8b8-4690-aa80-8d176f4f43a5','86496683-3bb9-4216-8d0a-92d272e53489','37eb47b4-e1d5-435b-a7fe-b21599dd4451','8a7462c2-a9db-4473-9417-7f19eeb72d35','0f9293e9-4f0f-4f0a-a54c-a6ef957fda16','67dac7ec-573a-4554-90fd-60ced4a43cfb','553343fa-8b25-4eef-ad3b-2e341475be0f','5f887a96-6b20-423f-b343-1ffe6e107efe','044049cf-f107-4e13-adb2-4a24688b0324','a650f992-b804-4fc2-bf11-aed3122bb3b0','797ce1e6-2ff6-4169-9646-ead66416828c','0e8e9463-4586-4259-8fde-d61a9acab6fc','7bc05df3-0165-4702-a2f1-7778bdfbbe30','edc2c16f-7aa2-45af-99ec-87a8a3474145','a4055618-6b40-4892-b416-fb67800c6f42','7de50d0f-cf60-4d9a-9911-e7297b0c68d3','4cd4a66a-18db-4799-976f-6f2ba3625d52','6679aaba-50bd-4d62-a769-633e0afa698c','39577d75-02fd-458e-a878-f1343a24c6ce','1f059b29-1ce8-49b5-82b0-a0f283c7c00e','74d9d534-78ba-4315-9e6c-1fc6a3892323','c52da944-d290-46ec-8e79-59ec4c64313e','cf3da656-6cae-49e2-ad90-adfd9443d99f','7150f601-7b9a-4795-badc-d0d3afa0dacd','9324e91c-2ac0-4dc2-85f6-cd49a21b2cd1','bcfeda08-2257-42a7-bac9-ca1dcb79f179','d21a6a4e-6e04-4487-980d-4464076a7aec','bf21ac76-554c-4920-87b2-3ca073f36b18','78b6a32c-b4e6-446e-9790-86ebd4a0b874','741f23a3-31cc-45da-9ada-2e83d94baf61','412e9157-f62a-4a16-9205-8576bff3477e','ec166bed-8aa9-4f35-9c0e-ed46b5dd921f','c814b634-ed86-4515-beca-206ecfca61f9','958eabad-6a3e-4d22-ba0a-d81449d453b1','3cd04505-9ed3-4c68-a29a-21b78590afd1','047a8da5-2523-46f4-93c4-684829dcdbfc','41af5cfa-1179-4c6a-9c5d-de3826a38159','7600c37d-610d-4f81-972c-d16e9b872afa','3e6b666c-08fb-4782-b03f-c0e51a900d71','7e15b283-292f-4c97-ac10-711eb4ea6187','061cfae8-7245-4909-bf36-789fb12d4189','3c58f62b-da9a-4f62-9060-d1fb30a21554','2fa89eb3-2472-45f9-9b5e-5b6b4cbe5b5d','4e2f9295-77d7-42a7-bc97-0cef1915776d','1373a41b-0855-42bb-81e2-49cb72be527e','ae5ee9c2-d7e8-4759-97b0-72e09e88c855','28d2d0ea-d6d2-482d-8fc2-7baf176f25ea','aacc97ae-9cb1-4f3d-a506-6c4ff11e2243','f4b4ac26-fb35-438f-905a-e142580d1bf9','c84ccf41-4436-4d50-a78c-9921baa3f812','e506f540-f4b2-49c9-9089-3fe86b0ae96e','23f0a0e5-012d-484b-bd23-c93c149e2cd0','51d7cb01-6d87-4f72-b52b-31d0434a49ea','88f853e7-5ab1-44db-b5f8-1f2510882f2e','13e26737-7c2a-4c6a-83f7-6d6742791392','a68af183-df7b-40a9-8b99-1565b43ee04c','3e626bed-de4a-4caf-8b39-fb3ee0c7a41a','949074d9-77d1-473f-b2ea-b0aa3947a33e','6a0dfbe7-b719-426a-ad3c-c0c6f10cc46c','d1531967-133c-44c4-8cc7-1bf6a8c708b0','c70f8e0d-b054-40e7-8c0e-72674fff0976','2dd32af7-5691-4480-ae82-8cec4969f78e','297705b5-3ac9-417a-945f-1a0f52828795','1e541212-7b91-493b-b92f-6cea87311449','3f4e6508-fa0f-42da-ad89-c00fbf3c9154','bff5a443-f2cd-4ce7-9cd8-ba45696debc7','fe6f0d54-413c-4956-9c02-5efe06178db5','b7dd8b00-2cf9-4610-a6ff-81893b4418e9','b3d3f219-e784-43e5-9dec-bba4e50c11fd','7472f1d9-e796-4569-a0cd-845323c5bf9c','d0f12409-33d6-4ed6-a86e-ce1120df3534','54d4991c-0e8e-4009-9269-f9e5d665dd26','e1eeeb7a-d9af-42d4-b53d-46699e7bd428','e63b8bda-8195-4b2c-ac47-8144e79a2d08','1efc24e8-cb10-4e2b-a94f-f5b3cd475888','a3b1f1c1-3541-4b67-8b1d-b72ea015c710','0e4057dc-c4db-4fe3-b841-ed6dff3cefbc','0051c253-0c92-423c-9ecf-7e6b8286868b','ee48bff6-168b-47e0-89a8-9569d332f9ab','07aaf2e0-1969-4220-9eae-0d952765f574','8a56b938-2cf3-490a-960e-e554477c313c','a5765093-3925-49bf-88f6-76423add5a99','4f9a7d4f-f63e-486f-9824-6bf8f1c9d61b','13043342-b99b-4cdc-a687-2bdd9b52e074','61b4cec4-65a3-4b2d-a6df-997872568347','81748035-e04e-4281-a6ff-bf57b3405690','5bfafbd1-7a8b-47b0-b7bc-093e9511e564','e34d6026-453c-4aec-91ea-024471ea2765','b62b3707-6c13-4536-b129-74a3429ef7ed','2de7b0e3-5e24-48f9-857b-11e4952a8eb7','0420b0af-5160-48d6-8bd9-dddfedeeb4d1','62b58368-3012-48b9-ada3-c71284bd91a8','0b5f14e9-321a-4d82-bba2-09c93c48d8ec','908e8151-5e37-4ac3-9477-9447e7e7364b','dfe28daa-77ae-49c9-b180-bbad1935e4ad','340c2a15-8a0c-4315-b9a1-3d3e29a66789','4fb31c4a-8297-487e-b441-41b512629321','03405882-2447-4bf1-8a56-f0d57791bc72','bc8e4b24-5680-4327-8bca-fa03d1d77b5a','a7b87bdd-0a18-4493-bdbe-813df80ac374','d75db7d9-8170-4f49-90c3-1bc39fd11193','8f47959c-c26f-4fd9-9449-a292a2b14bbd','e4d42b9e-58d6-4e79-a105-3105ab0a5b82','6b114c38-c7e2-40df-b1c8-ed032033c7b1','15b6d659-a226-4858-95e8-2abd948b2c9b','b7b546b9-c631-432a-bb4f-88387805b822','4c038fea-cf28-4537-a781-e43687aa4058','e2d68c66-4659-416c-9d45-fb9567d1d457','210965b6-e8c6-443c-b6eb-7ffdad60b2fe','e453c6ce-547b-4fb3-b762-ebf1f6590b2e','8f504a65-8cec-4f8f-b84e-89d6f12ae6d8','aec7e454-38a8-4320-9553-d720a0eb4c64','62d38d6a-16cc-443a-a54f-58555749d22f','444c14e2-e6ae-45f5-a083-18e8723a509e','b4578829-c8d2-42cd-984a-a110080a6a8c','321d8e7a-0310-49da-8e17-f0d976352b0e','2a00e2bb-3321-4053-b983-c589100b315a','0eaccc3e-b461-4b83-9854-ba3226cfd3d0','6a8cc741-5c8b-4132-a4f5-ecb019b5c226','b2849d62-4d6d-4803-be74-1e3de09ba978','e595e813-0526-46a7-8d9a-9776b5dc3055','312a5a76-c7aa-4f3d-b59f-765e205b53c4','b89776f5-b497-4199-beae-5053b0070000','d8236336-f4a1-4bc1-b99e-1962bed4dfe5','287d507a-1606-4438-8c27-ef11322b79ea','af3a2d60-3b5a-4d7b-bbf4-6827afd64871','40fabadb-0282-44fb-9a68-357ffd24f666','f703e20a-854b-4ab0-bd4d-359fdb49ab56','d9ca8476-ce95-4ba6-b6fb-c6a626574887','bcabfe4b-6f7a-4380-a340-7f0f750592b6','2fbc740c-ab6a-4f37-98b0-38459c5e6f24','85f6f680-657b-418d-8464-0626a538f2c4','2e4efa61-f8eb-4f3a-bff2-581bac99c0b5','5b9ee362-1928-42b7-bca2-bda7275a1257','8e178b5a-58c9-4c14-b445-5757d1ef1445','c151f1cd-19f0-486d-9082-0de7826d696b','98d3a34f-9ce4-42b9-9c83-7e4cc4b612df','72fe620e-3cc9-4eb0-bdad-3f79b9d70bee','fc9f18db-5e53-48ef-8f01-ba377140a6fa','cf1f3204-44c4-4a9e-bec5-ff1bfb905ea9','0ace9446-6a3f-4dec-b00f-6fa711015131','7457cb93-2e12-4735-9125-3a6e172397c4','8a172f21-005c-4a85-848f-211b3f585b7b','68c158c6-f4d5-4f34-a643-e7aab5781af1','6b987bad-7c9c-4a09-813b-30303fd867a9','326ab8c2-a3e1-4c83-be55-6ff1bbf890e1','c51096d3-29e1-4743-98e3-96483f496b83','5c5f6f70-0993-437e-b3d6-e22ab3d1b77b','328db4e6-cab5-4f02-81f3-838a96dd68c3','f2a0c069-119f-45c4-b491-474c3a12742b','44c96905-1a4a-4f84-8c39-eb0d573c349a','55bd8fd7-59a5-4440-9271-69b71e608afe','c7606408-ee53-44c0-a370-e0cb144d8362','9d1846f0-a102-4403-ae83-893f7c3de2bd','1537c48d-8e21-42fe-8297-4c973c8bfe74','81ac8053-cfc6-4c57-9b1b-c2f750ca6a0b','5766f516-b9ff-4724-b868-57fed1c8ee13','6cec263a-8282-4325-a6a9-8955cd193662','e5d994f3-39f9-4d72-8d0e-3aa47164a573','347e37e2-1a40-41e2-a163-9664aa13a9ea','67d35383-b553-4b5a-9fdd-59a6e6333690','b1acc20d-ca1b-41e0-b06e-372955247c77','e777e570-8d00-4d55-9583-646aa3ec9ba3','46c5491e-f598-485b-bd03-9b852e4d7c70','88c630ec-7785-401c-9256-d18e457e1b9a','19341d33-22c1-45eb-81a7-30a155633078','237c984b-f253-4160-afac-5174550224b2','5656ec51-d70b-42cc-b919-b54d391fe6a1','790c0bc5-1918-493f-9077-9027dca82084','ca87e4ab-e34d-4b11-a194-7f41fd403abb','a5988538-52ad-46b1-98b8-ef1993050aec','39a643ba-218b-44a6-bd57-53c21db08d3a','56ca0c0c-d1d7-4c2a-a49e-095a3aecb4c3','470b6c46-f3b2-4d14-92dd-f0612820d4ea','6470930c-2721-40a9-8235-98be5773eab2','95be8c33-91d9-4718-8533-af05538e1b57','16b459cc-1775-4d7d-b996-fccd9dd0b9d1','aea1d812-5db6-499c-b953-215a74da3e0d','57db31ed-33fd-444c-b300-23a90120cb55','53e620a6-b4a5-4862-bc3f-0d57a403deb8','4518d4e6-c6ac-43ab-80ec-77c948200f4d','8b005c1e-5a31-42a5-85e9-8e6c44418425','c8070860-436e-4967-a010-87cfdf25767b','7c1e0780-9120-4d32-814c-bf05d4bf0a40','64c7ecbe-efea-44fc-ae6a-063f777704ba','58fb2626-1094-4d16-aedd-86f0d3396125','bc99cf8f-a23e-4ccf-81d7-ec17406750fa','5567bd6f-d9f6-460d-ace0-ff6d53dfdd92','3558859c-4d1b-4a3c-9968-c2cd1d856e99','89712c6c-a8a3-48df-bf80-844e6a5bf24a','a64d376a-5506-45c4-aaea-566b9ab098ce','7f7068ad-616a-4c33-a780-e0e391f8c175','eb0c1975-66a2-4629-9df9-68fea3176e71','7df38375-51e2-4e3a-b0c8-97b731006197','157ce15e-e1a3-47b2-a3d2-4a639ba9c89d','d0b4a99c-1503-4a69-9eab-74f47d34bd93','c2b7e2f2-3d8f-447a-a7e2-875d707a58bc','7eeedc99-677c-4c90-a79c-e9768b7ae427','fdf96edc-a28c-46e0-85e2-944301e5bae6','dcd1db04-be1f-499d-a82c-b600136d541a','f9120583-9771-4487-8c5f-5c8ac0f1987e','143307ec-4e31-47cf-baca-ade7a4a682fc','d6962071-a956-4e45-ad3f-b5db254e421d','97c065c0-43d1-42b4-bd35-4743b50b390a','c4695b40-7e3f-4141-b15a-a8bc49f11fb9','9fd0b58a-36e6-49b9-9b0e-a32e58d69e50','eda9f9cd-c7de-4244-a798-589f50a256c6','251c3616-5b68-4ad2-a87c-c5309fe6c446','bb123eaf-018b-400d-96ad-de176bc66c51','48a246ad-3e35-4954-87fb-d4ed92949b20','7b915fa9-a7f2-422d-8836-74fb85ba12b3','a62f3a25-bd4c-49c7-a6e8-eae92f71c5eb','360d4082-38aa-4179-a948-b47ce148a40f','d4ec8056-0cdf-4878-9055-dffc8ce29820','e98cc944-dbb4-4e3b-93d5-5bf73b3317f1','9b053b93-eabc-491d-9ab7-664c6c3bb037','d2c39ca0-9a5c-4553-927c-105ca980be51','7fcc357e-46dd-4dd9-891c-a33aab5b590f','9a010a1b-75fc-4114-a565-e25c9e3e0352','1e3d7d8a-2eb0-4ca8-af6c-723a1b690352','e25a3ba5-7704-4ef8-be82-bce2f3d954e4','d2e35b00-06ea-4502-9f2a-0833c8324e22','c5a58015-90a6-42bd-af6a-9b6abd49938b','98a4844a-2a6b-4df1-9023-1ec9a6d5e595','a5288757-ec7c-4bee-a0ad-6a973ae0a17d','30926b72-bc51-4531-b150-8f69fe781e18','05f3fc92-d549-46f9-b2df-f18eff1af6d6','0f1e9120-fb26-4f49-8212-48fa523f5d81','40e88b9c-0de3-40cb-bf75-b16bed8fdd23','45375707-3db4-498d-8090-c744bdd1015e','22bcee40-e57f-453e-995d-c490187f268c','02faaa45-f92a-4a91-a557-3aaaa84ad118','83934b20-1f6b-4af8-a7f0-fcfdd518f344','aa1d7ef3-47a8-45b1-a9cc-e5a0175814f5','dcbe7466-7ebc-49af-94db-3542d595aef0','8b343291-3470-4055-bd26-0e2db9b2a64e','6c414344-7aee-496c-b6a0-83852a1cd737','52511fc5-8193-4547-b77a-aeec1f30af7e','8452e06f-0ac7-4c96-9c07-f867b9d6e143','4ec54d1e-a408-42a9-b572-e4ea4d8da8fc','455dd85a-14f8-46b7-965e-f4c4db4a5cbf','684abee6-e554-49b4-9acf-4d86986b3765','6e3356b5-b04d-4d72-9859-10f31b66f742','6b042d63-2b7a-456a-a37f-4ec1478b8fda','cf639e62-02f7-4737-b1ed-497c7d7d9b67','504f84d4-0502-4ca0-9479-5fdc45fb279a','be29d80a-e0df-42a0-8393-6b2784b7ef0a','4bf04e7d-775c-4c4f-87db-2abe2530ab47','ad492cb6-c852-4c99-a152-c1664b82e21d','05890417-a898-48fa-9e9d-74c32129da05','19a30205-b98b-43c2-8147-2319bc2e58fb','fdb8c987-f23a-42f4-b54a-73374028b625','0545c81b-a601-4ebf-bf7c-a06efb75189f','26b85df2-656c-4a04-b5ff-5454e2a3bf36','c411ab4e-5faf-4ad4-ab9c-99d2e0534b7c','e0bec569-b8a6-4dd9-ac85-fdfc557d1644','898ef14d-be4f-4117-8ec9-3e3543bcb1ef','aea0625e-b058-4927-9fd5-11de4248b577','e70351de-0dce-4b4b-8c80-51dc95963c83','eef7c070-952a-4476-86e3-54709b6ab59c','fa4232c5-7f5d-4deb-8607-f243c9601359','64e4fdc2-0b17-4471-9f31-ffaf230bd574','adbd5906-9cdc-4cb1-a9d5-b1225a7e7de3','0f322c6b-1bb9-418c-97c9-5ab714275f16','1b561f05-f74e-4ef4-9464-afe3aaed99d9','0a7035a1-0caf-4cd4-903c-e363b089b1d4','ccea5020-a999-472d-a643-72e1bf6b3da1','4a1c77db-6039-4169-a45f-5ef866cdd2d5','8273181c-b2e5-473f-ab53-e5ac35a47688','a122ab7f-b91f-4966-8e55-c7fc68886702','56d5557d-faae-4e36-a067-b27f99d5a328','30ebbb19-32e0-4016-97c5-cfa9b76d55b6','e0996433-dcd6-4b00-bf89-5239c600b01c','0b124add-10cd-4165-b8f3-e6639fe36194','3cc6dd69-65fd-439e-870f-dd821837d572','442dab3a-5114-4ce6-adb0-3d743813fc50','43851f0c-f5a3-4dd1-947b-716870e6b11c','c96393f4-7d80-42e0-96da-68985a6dea24','6dcc4b1f-ef62-485b-a579-94a0ced17c30','68c38803-eead-4877-86f4-45107397c57b','3da2eb58-d35e-4607-91ac-2f37bde94179','280b2dfb-d3d0-49ba-8592-7909c1529a8f','c19ea747-87b5-464f-afe0-a0db00868637','cbbce55c-a46d-47af-a4f7-855df688a1b7','eab0285b-524c-42b2-ae23-74ed0ffd5484','574c6df8-7715-4365-93d2-12a47385d01d','5f67383f-9097-4412-bb0f-21b0adfdc3f0','7fe670be-e89f-4ccf-acf6-fd6a3a610958','8ec913d0-0665-40b3-a0de-96974191b15e','d83a94d8-dd4a-4463-b8e3-12db84babb8a','685af08a-2888-4183-a961-fe5968beef90','3f36f44e-58b6-4622-8b2e-00610c22c292','9d7a73b6-a253-41fc-bf60-665e5720ad47','32413399-0c32-47c2-8b49-5772f3c3b12b','1cb5d317-551a-40fb-a1d6-c21706910344','0f249fc7-ce89-4a1c-b2b3-0f614cbed6fd','cdf1c2a9-3631-4a74-b5c6-89c864cba2a7','cf40c8c1-87d1-4a11-8b7c-7b73c7995750','14449a57-2277-4bb2-bfe0-7b55a4bbba4e','c69216af-b1e2-4c9c-8e06-08794d3930d2','57393673-32e8-406b-adfb-061f50e28249','b066ddac-ce46-4e38-8696-fda36a70cdcd','80900154-6849-4a42-a572-fa9af619c13c','2a2a56eb-af7c-4029-90eb-862209dab464','2adb4a8e-b5db-41fa-b109-cc21340a2521','18622c78-5884-45b6-b5f5-26c7d472787f','7cf5ac2f-2c7d-4cf4-aab2-21ec0054850a','799d8de8-fbdd-4da1-812c-b055f8cfb474','e5caf285-44bf-4128-9a5a-abc1da3c292b','f7f158f3-3857-4845-9b48-99ae1dcc0fd2','592e2ed2-8f70-4b68-9e9a-99547089bfda','072efc64-70ce-4e48-ad0b-0ee4af7f4a9f','e51ee2f8-22dd-4db1-9fc0-fffb5a53317e','430b0bc6-c71f-45ce-af97-a920bc21e804','bd2617e1-081a-416c-85fd-19a6cfc7f6cf','3f522dc8-58d2-479a-8468-f8759306aa8b','02c639f3-d2de-49d6-a401-5a8261789c18','5e1904d7-4b73-4a54-ba2f-22749fcc2d02','7a642b4b-026c-4237-8505-27a79507b738','250c0fba-931d-453c-9e92-34071d1d583b','a185eb86-2c91-403e-b652-fcea4d2d4ee5','f1edd906-d8c6-4479-a588-eac801ffa89e','687671cb-0533-408e-b909-7d8bfa6c6cf1','409ece50-346d-4626-8a39-ab5566c3165d','df0a91da-6660-4e3d-bd56-9ede09706f37','85df3b50-803b-4916-9d41-9c1a28932cc1','227ac283-70d5-4880-bc9f-25fa7216557f','f986a82f-5f34-417d-ba92-4c2a7b73122e','74f48d7d-f9be-4ce2-ae04-0e4d4da9f9bc','afc210c4-d1d4-4063-a0d4-a81e7af4792e','0ef27249-f40f-486e-ac47-ca89442688ee','483e94a0-273e-49c8-98b0-79c91e9741b8','bd695f32-9476-42b5-97ec-fb6705f26259','ac5ed0b2-9b47-4b6f-a515-57d11f5adec2','87771efc-8c2d-428b-9477-13d253e45b50','39cc41e0-54d3-49f1-8e00-872c0fdbc21c','14339b14-539b-4a01-99da-2130a4f38449','f69a32bd-d1c7-4a0e-92ed-ff9ce6fe8160','e3f823d5-3358-4435-a6f6-3c93fbeadc1f','444c73d8-556d-4a7d-8272-ee188c89818b','f71cbb5f-7e85-430e-a20b-075ec986c75b','6c59f779-80f0-40a7-b9da-f60791b3b979','41645643-3d67-4129-9935-5d6c8b9590ee','1cb2e749-75ff-413b-be56-19beb12873a4','21b597fe-cb91-49f6-b072-0240ce3845c6','52353fd3-1a91-4249-a4f8-2322ca945490','bd682656-3875-4cf6-8137-1d39cb8ad834','e48a496d-6ebc-4f23-a93e-c732e489c06a','1d46d0d8-c260-4bff-8deb-7d312fd8b2fb','2f1fff16-9c6f-48b4-b196-190dc3adde79','7c84f7e3-ce8c-4c5b-8cf7-295bf0f2fba9','eb6dd016-6fdb-46cf-846c-7ff5b513cd2f','7a4b5505-315f-4bb3-a3fa-d9c6b3865621','b836ab4b-7fa6-4af2-9ca9-388978b14ab3','890a9667-3e9d-4f64-8e32-7039f2495778','059cd936-a575-4fc0-9842-2c5178218a2c','b2c4fd25-40ca-4ae6-91a5-9334eb33ed5d','6f7ba61a-90b1-4aae-8089-d07695aa9d77','a1eed484-4590-4ebf-ae7f-ef2457153841','246ebf86-e9d9-4870-804c-3e62717e917b','43efe5c4-ef05-4fbb-9d18-7fc501ba2936','919e82a2-907c-428f-bb2d-b1b2abd10466','b19af3cd-64e0-4c35-a7f1-39edbff31e3b','8593d24b-4d6f-470b-b69d-c44563f39c33','7087afb1-aa9c-489c-92e8-c580ce00de03','20f79201-52fa-4cd6-b9d2-b9c3ae376c35','0e7d3f2f-3774-4b86-bb46-e29cf4ca4d16','12e6ad7c-1e2c-419d-b51b-2df56de8bc72','85d5ec94-2008-4ed8-b630-b2a2e81d0231','755e091b-a7f0-4573-89a1-b6e4980d0432','bf8b3168-0ecc-49df-bd06-7cb1826e11cd','8908c011-65a3-4e64-bf36-85732940ca08','6fe61f1e-a3e5-4bd6-92f5-07383f8a47bc','31ded3fa-2b80-430f-8a30-2c02e2a44ec3','cc3a52b7-55f2-4637-bf5a-834b5511ffad','a0f6b9ec-b49c-4c54-9fbf-d3f081a07566','f9b63713-c427-4faa-a0ae-ea8319043441','5d996f1c-7210-450f-b673-b5af67e18f33','b4a6aaf1-66f7-4a3e-b12d-a0c8b2ce81a3','316a85da-9af0-41aa-b33d-d272414acbaf','a59d5609-be61-4f17-9243-a73ce849c049','1015dd75-ca53-4dd8-b183-cd07bf860c10','c0e7a8fa-a3aa-4732-9dc0-7a8af0ebe49b','6b316bb1-6f35-4493-8610-679762292490','e92338fe-adf8-4eb3-9b99-d57d86e4f6cd','070dec1b-add6-4822-bf84-d2b2283bea70','cdd1744a-7962-4e39-9943-b59a2cc74e68','9f62e6eb-a3a0-470b-8581-95fb33452193','9007a1ce-aeaf-4775-b295-839042c46dbf','f39fd97f-4016-4732-a1db-b205876fb21e','f4e83cfd-01a1-49ac-8012-474a93fd720b','253d2fe4-c0f5-4680-be3d-a76d6c870864','11ba432e-573f-4294-8fc8-2d53b771c49a','437e7d7f-0494-4c04-af66-da1df7d6af61','8cbd13cf-23b8-4dba-a03a-f7905f5250c0','34215cc6-43a6-4b0c-b01c-acda13c10a0f','39f84ca7-0a5b-43e9-8f82-bc22cfa8edc5','ce6cf416-a7c4-42f9-9015-ddbbb379b92e','73a48187-f93b-4b2b-a829-9b6d09dcea52','f7d6e29f-69cb-4eba-afa9-333ca41bb7ed','28b13211-7c5d-456c-82e2-eefd5a470c9c','f6460d32-a306-427b-aef8-6f9bee92fca0','2d00330f-bdcf-40ce-9ddc-4cff778cdd8a','226ac646-7b0d-4a81-bf01-bf370554678f','bd4a3ea0-5d7f-43d2-96b7-15577942259c','2bdeaac4-6efb-4200-a4a5-083450b47b55','14a517ea-a669-4696-ad20-9b953b5ffba5','2a6c72a9-e24a-4e60-a485-24c7b555fbcb','ad4f8a12-9047-462b-84f3-997f90e11aef','da1b3f28-20eb-4c24-b435-d174925cdc7f','56324dee-c92a-4e1b-8c61-096bb75a9f36','1a3510d3-ac6d-4a51-a032-a4ed75123202','234b0071-e093-4801-9314-cccbc1788139','d45e34db-2c0b-43c6-8475-dce741fd1cb6','aa3127f5-6ebe-40d7-a64f-a29e6acd4767','16896ef7-789b-439b-b398-7d879d646645','706ea8c0-fcb8-41cc-acd3-aab54df6d2a1','d25d6048-cf9b-4651-a70d-bbc66836ed58','b6176936-c938-49b8-b997-ab5b8fe4ddfb','4e1eb252-1be8-4802-8d8b-82265ba30d10','452c1123-8f5a-4d6e-bade-4832bb3f7c9b','ed05e973-6240-4306-8e50-b5fe3dbed4a7','7a24bb5b-707b-42b9-b7e4-cb5973411e68','437f8f2f-16a4-4c52-a893-89644920b64a','388e0e3b-3f60-45ac-8a5c-92c940d1c229','1f74a4fc-10ae-4c9d-9dbc-096e264e08e2','efe79b59-ae41-4144-bd71-811dee0a02e0','a9c13b31-6238-4c9f-8bf6-a3493b1ebc55','f73f2594-4aea-4286-b334-5f0034ba6268','7315c6d4-9a6a-4cbb-93d2-f7c5fcc2ec81','4d3da143-64d4-4607-b9ec-5315674cae5f','1e08ef33-f38c-4578-be02-e91b99b23d11','5682fe1c-57f3-4340-b1c2-6eae0b9be6f6','ef1c221e-05ce-45de-ae70-4c0cef45db43','21d34bc8-0307-45b8-810e-7ba594c684d5','a0cc5433-ba3e-499c-bc18-9c539b8bfc47','aec15087-691b-4865-8b46-189268394a62','150462fa-d581-481e-87a1-8aefc606e4c4','e1d5d4e4-1d1b-4fa6-9bc1-aaaec7c94c9d','8c308df3-a8b6-4b02-b401-d879eb480452','de89142d-4810-4014-a9b1-ea2def1b498d','210dd1ad-ceeb-4926-aff7-dd45e2600d77','d1ca65f0-feb9-4945-9a3e-2ba07890f86c','fe8035d5-2098-46b7-81c4-7ea9a58bbf36','3239ab2d-6ea0-4880-aa81-6c3d4521502f','60f3cf6d-a32f-4f62-9b17-234d2fe5effe','d7a0d16f-729e-47a0-9c4f-e649ef172342','8774a4bf-5c65-4413-9110-2878b2e31ff8','1e415d1d-f0cc-4ed2-84e2-e2869833dede','432edbb4-4c31-491a-9a6a-ad8f01b0ffbb','2a4f36e5-dc2f-4928-b6b9-5dfac460bed9','f5055404-7b9d-4e25-a4d8-e276dd014818','cb268260-ed03-419d-909f-fdf7f6f5351e','560bff01-30f4-47e6-adda-1fb0c219031f','905fbb2e-8a44-470a-a024-fbc352ad0fb3','e9451913-8fd6-4104-bf2c-366cd3f8056d','1655d3cc-de14-48e1-9222-34287b63650f','ab943067-4f86-4a8e-955f-e9ce21bc0582','4d11eaea-163a-4543-a05e-ffd4f66ac423','f017b68d-631c-4208-83c0-2f017fbb0657','2a78aed6-3044-4602-a4bd-ee628fcff655','34689905-3226-4aef-81a7-5658e1c6c386','2ba464a2-dd2b-46aa-815e-ffd24a065a52','2b4b1022-bce9-41df-b926-1b72b060f87c','041ad3dd-7638-4a14-b378-6dee2e604cd6','73e15eeb-b7f6-49e2-8442-83ff807543d1','8ef54230-a869-41e9-85ad-434c0a9b102d','cfa2cebf-432f-49ee-9cf2-1af14cba1a69','eaa2cae6-9968-4cac-b851-1c4a78c61211','0c64176b-0046-4e82-8210-df31f390eae0','70066ab4-c86c-4da8-b315-5700f942da50','0f76fffe-9f66-4c7b-9f0d-a15a0fa3185c','6c451783-f4a0-4383-990c-27dc84b51acf','f280fddf-1706-4ff3-bc70-136e0b377253','715a5461-0f13-44ce-a7ad-5b34f6ba73cd','ec6d72d4-3c4d-4329-b7bc-c4025f2d417d','c8f11fcd-6278-45e3-af75-0a289d71ce9b','8baca3e7-e219-4d9d-b4a0-c49bb40f889a','7812b1f7-52b6-4e9f-ad98-91034ae98f22','6349328c-6cd4-4946-a021-799ae406419c','b1e9e332-3bff-454c-bd0f-a66fbe1a6203','f9c18979-592c-40f3-8e2a-1b76311f9a3c','3a799c4c-b49c-46c6-a55b-ac18c5725d82','8697930a-4a55-4e62-acc9-119d4b13f36c','e8b2690b-40bd-412b-a171-e74ae481c32f','e0582500-86d4-4c67-a4a8-e8dc755428e2','309b8e41-a53d-4ee0-8fe4-f4ce189f890d','91d02cd5-31e5-4626-bacf-5160d50a50e2','3f77dd04-c594-4695-a8be-897d82ec5290','452cf6b8-1fd3-4678-b955-620f90db9f09','c96c6bb3-cf8f-47ef-9b3f-0eed7eda4a58','a45ca9a4-6ac9-4e7f-8737-d67db9ef00da','5998eaa6-f730-49db-a1fa-e33edb68910f','11768f61-204d-46bc-9801-e699c69104f3','0f387278-be6c-471a-a851-74da5bb87c8d','571a1e72-75ea-4f23-baad-b70b0dbdbe26','ded269c1-a64f-4ee1-b607-8dae1c1e9108','cc14660d-92cc-4e68-bb61-d6484d536bea','1c6153ee-5514-4bfb-a835-8760984f2635','57829722-09ba-4407-8b32-42d170efd75b','ba998f3d-c177-4d48-8bd4-bb6f92f166b2','2c0bb692-0df6-4fb6-886c-4a337cea48ef','8b16c507-ed55-40c9-af9c-495ac0cb5547','d87cba04-f876-4fd2-986d-e2c352f2a16e','31b01277-e92d-458b-a1cf-34535cdb10bd','62fac2c3-c7cd-43b2-9d84-d7be81ebb1e4','a446708e-ba47-4666-982c-a49fcf52f8f0','0524799c-6fdd-4449-9ddb-0576f97b935d','279ce3aa-98da-4350-87d3-7442f87c51c4','9d021934-2c18-4ecc-99bd-1c0f5694f6f1','6a14efe6-d1c3-4230-a902-b7c472d09315','016aa589-6976-4d29-ba56-43376ee853be','3466b459-81fe-471b-acce-ec73b797ebf3','2b272593-f14c-45fa-97c2-e80dfdc023e4','9d9b617c-47ac-4982-a6c6-e73d346c34ff','6bc0181c-5f59-406f-b159-bdc0e55b94f9','8b8dafe9-9952-486b-99be-9a43bdc3a0c3','f2161de6-1a47-46d5-bf3f-feaf07a878bd','2ff07209-7571-4f0e-904b-b0ea5c9389d4','9b0bb1e8-7f93-44e0-a0ec-3a7c6b372c9e','cfa88589-47ba-4c0e-af1b-f54f2f18954a','0a12d044-7cc8-41f9-ab04-dff3e6681282','2dda85f9-aa5c-458c-80e6-b0018149ef39','5757fb96-ed23-439f-a475-1cb6e0364e03','99cde64b-147f-49a9-aa59-dfabe67c3774','57e04deb-b520-42fc-a746-d3bf01f62ed7','e8e4b75e-865f-423a-9b0b-88eefff2fbd8','08d86e52-4ce3-4b26-bad1-99b29764b3ff','816a7c4a-75e2-4bd7-8778-ad95c870e781','7a62ec21-bece-48b1-9e76-a47eea3aaa99','ed1562e2-aee3-44c5-8a91-fb285d94a0d9','9e88add2-a51c-4f54-a0ea-86666f23a015','438c7bea-08d9-4333-b8c9-8c467d02103a','e3cbd4a0-b4d2-4f58-867d-2aa6024211db','fd8564d0-a010-482e-bc0f-fcd77c130430','ae484eb2-2e3c-4915-9cb3-c9582d56ff63','21e78b65-610e-441e-a4f5-5c0adf5b5726','a43f2fe7-4766-4db2-9bf7-27a7d0c12fa2','7755d59a-6c93-4c4c-88fd-2f31d0360c7e','c049d84e-77cb-4e58-8be6-9bd382b46b76','9eee8a91-a5b2-42bb-898f-899d4b32b349','fd33a66c-a4c8-43cb-a536-6282571b6bf5','c74e4650-e81a-4ffe-a24e-8359d61b2dca','3e7c8b93-a35a-43e7-800f-16c782c7bf51','7d983c5e-c3a1-48f2-915d-17e725b0a45c','f730f58e-1645-4ecf-aa7c-a13c51f074d3','fae90a4b-444b-4f5d-a5da-0107f152adeb','00204970-095f-4c3c-a29c-933502dcbdee','d3a6186c-d91e-4d58-b2a2-8977c0dd3412','a31127ad-a1a6-4468-be47-13eb99c3b413','d6a7239d-4fc3-4f8a-ad15-b3db9d84662d','159692f4-e3e2-46a7-b15b-5f1af1111889','ec3331df-06b6-48f5-bbbb-c7b01e30ad35','4fba0a31-6e64-4e66-a74c-fba9c66bf82e','f5591185-6713-478c-80f3-424d1c9ebbb1','6b700c97-5505-494e-8a57-710b1a13ca92','d14a0864-5a17-48d0-b368-4739d28a0d0d','dadf918a-bc21-4101-a5eb-dda6040738a7','c2990ece-ea79-4eb7-b54d-e6afc5f6b0e3','1b900bf2-9563-4b88-8f5a-39d39e7e9dd9','add26f40-cbfa-4721-b48e-cc972981d880','8d498a9d-78cc-4263-9c83-008ed8a57d7e','1c953d2c-f6df-48b7-b271-1a88950059ff','8c17bd09-3922-43a5-8300-2dd50993de48','15a0a736-4af4-4c4a-9731-019fa4571ab7','aab8c1c2-5fc9-4c2c-a153-e3db95e3cd7d','91d67c68-d023-49a3-bd7b-e386cb8556dc','b6759936-59f3-4cfb-ab86-cf82bf5f39e8','f73235b9-d771-4eee-bca5-434d1c10a3f3','4f6d64b2-862e-4f9a-9f0a-e44101a41db9','ac1aca22-19f3-4478-aa83-4c25d9171c6b','aa6dc09f-755d-485a-95d6-3f246288cded','0b7372cc-c4f8-4f5e-a930-ca232ef85f31'}}),'106708',struct('BlockId','2af4b13e-36e7-4c9a-aaaa-1b2c842c5568','SignalIds',{{'721a1796-11cf-41b0-9af6-8a1d2139646f','cc50166c-4977-42e2-b10f-7eb72e0a12a3','4104cee0-7459-45be-95f2-584bf3283c47','2ac8c89a-613b-48e7-904a-3674701c4e6f','11bff659-a936-47b0-b20d-98d8cc58e70a','2d60f184-37d7-4fe3-b0a9-b77988b9cc9d','efbcfbc8-5552-4bfb-9893-b5e291e13bf3','ecfc2b0e-31a6-4b8f-8b52-61e9e0cd5929','01be0e75-db0a-4eb0-b71b-269573412f54','9c48adca-f804-4bf3-b128-d01daa909d21','ee7d80cb-8b51-407e-a736-04711948415b'}}),'106709',struct('BlockId','771209c6-0331-4b62-a043-30f8098ff88c','SignalIds',{{'947f247d-f903-4bdc-b849-ff4c6f3975b2','a5b6e8f7-a821-4927-aa40-631157b17a08','a7c596cc-14d1-4435-a66d-d7dda8a7aeaa','af53ae0a-a857-48d9-9d3d-126345c0c488','7921379b-0c05-4b9d-9d78-36567de47601','58d50734-8489-46b0-8f07-802a42684c35','fe6c0aba-9b9c-4beb-b1e5-ab312af11a83','46ee5e49-d09c-4b2a-8f73-e3572d288a46','c577708a-af56-4d8c-8132-6fdf1884d5c0','71ed6c3d-7ab4-4d57-8af2-2ce511eb3973','308ce60a-ba64-49a5-873a-0e4e9c953d65','8329b7c8-d729-407a-b0f9-df1e5232512c','861a5dff-87a8-4d97-a9e2-d82d1644748e','77fb1827-738e-4ebd-9526-ab95b38267a3','b88a87e3-c06b-4b35-b4a6-b89dbedc4e34','e3dfaaba-85c4-4f1a-af11-4f13b690a2f1','4902ad2d-7fb4-420b-9cfc-5b200bfd5779','b95f9309-f50f-4f11-8d41-4cc6ed67bcf7','ad75fd7e-854e-49c9-9314-5bc3f4f1e99c','b3b4414e-a2c9-448f-a915-ee39c358c32e','5bfa8792-fe4b-424e-8751-d8c285357b41','9911e365-4012-4515-b249-c46410c0ada2','00df9805-7dd0-42a1-a64d-47d7f40cb015','eadf7da1-d9df-4896-8e93-af71b4b90698','ad3207ee-dc7b-4c08-abf4-734c1ed59a35','64c1accb-3d96-43aa-b7c3-3a7a3db02ecf','a8fd6e62-10f5-4576-b319-363050333944','0ca89ada-bb63-41b0-933b-0b45c5037847','ad3c51cb-3426-47e6-bc45-6d3a4b1a34ec','7b4c0778-082f-454f-b7ce-e9ef3fd8f60b','0825af03-6c0b-4a9d-bd5b-bb31100ed4a2','dc083e1e-da61-4630-ac3c-5b26591b1c37','8ff03d27-6b11-461b-8930-8af8b5537743','f1197e53-7ec5-44c1-a518-e85913958f27','226e03db-8526-4641-9dff-207ef9c07b4f','549231d4-88d5-4679-880b-d3283fe8c76f','fe0822ca-6848-4f82-a9c9-3927e139026d','aa531f53-5bc9-4922-b0b2-216ac742c7a9','9e7febe4-4eca-4e3f-b042-b1a5df367a87','dea4c089-a939-4faf-a9b9-599cbf4b42e5','0339c28b-f471-4958-b922-ad12d6fce3aa','a358982d-d141-44ba-ac04-0b6bf17675dd','7d2302d3-a27c-43cb-9cf3-46d958429ef4','f5c6a838-7a73-4f9f-b6bf-fb84d08ec774','1811bc19-ed60-45ad-8e3a-72bdd1fda6f2','1a55ac86-a376-431f-aec2-178d163bc81e','f13eb4b6-8e33-40e3-895b-4b91ffe17f69'}}),'106710',struct('BlockId','5a0b0a57-2be6-4ba2-b173-79fe170af739','SignalIds',{{'9a0f6532-3145-49ca-86d9-ddb84d6d0fda','b97292d6-111a-4d0a-88fd-12db6a267f80','6e12df9a-f554-4d5e-b610-0887fd716bb1','7223a53e-ab2d-4171-90f3-440290ef4420','a661c362-ce75-4343-ac82-4b6d4b86578d','1ff98b4e-c938-4738-a79b-5a73025d1a4c','ce05e47a-63c8-4edc-8145-b89a853e3c30','89acfd9c-3f54-427c-bf22-cb6a6c644c6b','d1eb2300-21ae-48c2-a813-05aeffc97710','524b9f1f-c4b8-4f4d-af9f-fd744ac9fb43','320e06ff-2eb4-45b9-9e80-11be66660dad','7bba974f-a464-4b0e-bd9a-8098a3a3c8bd','a7f0a598-2c45-4d17-9439-1b9a54556b48','588e2c92-bd9f-4bfb-bb4d-4c7c7f9a13f5','6913d25c-8b90-41bd-a4d6-85bc12fbf6af','1fb69428-26d9-41cd-a6b9-3500cf59c079','29901998-81e6-4fa1-ac74-357bcd297848','3dce0260-36fc-40a7-bdd3-f32691d60c9b'}}),'106711',struct('BlockId','96929957-fd36-420f-858b-58092e5e4bf4','SignalIds',{{'0092404e-5dd6-45ad-a0bf-596ea91f0f4d','6213d160-e944-47aa-a425-f6a592953c8f','22af2b9f-6c18-4e1b-840f-4b9a6a070361','3a3bfc58-7487-4765-bcef-02837d2e51da','ed45aea1-bc6f-4863-b93b-011fef181245','3ae432be-614b-4839-b2f6-b2940821c299','6fe4561c-a69f-4f91-9b81-66aa41d096ce','9e9e673e-f11c-4df4-a133-084a57da8b22','95b534e8-56b7-4c61-9b8d-ee9c0f5d1049','fc607d97-b69f-417a-8459-a8bae001e7d6','a34edce8-e24c-4a41-a54a-ee3f69eb7ffa','b1a53c6a-7ce8-4ead-8b3d-f9c5af2c8ef4','e76fc831-b789-4630-b702-ae8e6af7a4a1','06be340a-b464-497b-9a8c-07bd9d33e05e','bfb60d51-2588-48ea-a51b-8427a61e2ff3','b6e719b6-2a60-4cd5-8e12-c0df62502af1','31b45a87-d953-4b2c-9da7-826cf68fc831','fc9eb14a-33d4-491c-9843-9261253ef45c','bfbda015-ceca-47dd-9ebc-3d41e555fcc2','36f9c4b5-4816-4941-8b4e-26a5d6dcbba6','a28f997a-000d-4777-b30b-8ce2b0bad8e4','3df6d612-976b-4e7d-9da2-2f5c4ba42bb0','d1a6d3b1-c3e3-4e90-9040-724b284a196b','05c170cd-3983-4f7b-b887-e134d9c746f2'}}),'106712',struct('BlockId','2e236ce5-85df-47e1-bf24-2be77924d264','SignalIds',{{'69aeb882-f5ab-4416-bd18-25119e1cd06e','33f82b7f-1ba9-4984-92ff-38fcf5080a5c','ef4f17c8-c5ba-4afd-b621-e6d1cd9e10ae','28a88deb-73de-445a-b668-91ba4fe52223','29af1e14-f559-4ec6-b329-6b819fead416','14b54d53-22b5-4503-8732-5aa2373f6151','1f8f0f47-b8dd-40c3-980c-b26de7eb2ebe','05716bea-1352-4a85-86bc-dcff0094b19e','b0130243-427f-4ba3-b5df-7b7bf8d852de','c4759555-3eb5-4986-8df8-9d30eab382f9','5c0da2e5-7a54-479b-a372-10e116241b88','c82b2403-c13a-4e31-8ed0-ba7ebc770253','e6180a45-e04f-46f0-bf7d-97e50ec35a8f','24009512-b765-451f-8d46-958db0d7403d','4f26e654-998a-41ed-aa86-fd4884b751ed','3ba32a68-420e-49e3-b1b4-49aef6e19e48','3b391fe4-b144-4b83-a0cb-c66bfa2826ae','fb204af8-2899-4357-8703-968a0409a0c3'}}),'106713',struct('BlockId','a577d8ec-67a4-4a08-b001-a0ad015f69d7','SignalIds',{{'208c5091-4226-41a7-a168-96399adbea46','413115f0-d42d-41fd-92dd-8df7b134cc3d','84ff84dc-ba84-473f-b31f-9e45da5ea22c','5d47181a-84d9-4474-8662-1ed983bb8cb0','39a1458a-906d-4c82-903e-13e1c5002d4b','7a7d2bc2-def5-4224-ae34-e00e23f2e146','25c5a3ef-65c1-4418-9e7b-378e914bc0a8','523acfaf-8d97-4374-aa6a-44bccdf0cfc5','2062d977-d2a3-4049-a6c0-bc4096983aee','1ee4f88a-61c7-49ca-87d0-11f529364b35','a263e2b6-84bd-4f65-b621-4677a1313ac6','5b0cb379-0328-47c9-a3d5-166df9c82728','2980d2ce-9474-4062-815d-99397b607a4a','a32c0566-ad1c-44f2-ba0b-84c151fe3a9c','946d5077-700d-4fa8-9ec8-69c3b283c147','d602acae-e85f-4ccf-bc56-99a87a18aebd','4cf799e9-f597-4280-906e-150175e3e65f','905a7dc3-9ef3-475c-a60e-8024e84d1639','aa3b823c-9dbd-47e8-90ed-4807d5b8545c','4007bd37-00eb-4c8f-91eb-f389e9b21f9b','a20fe91b-e6da-45d7-ac1f-3fa94bc67be7','e9f7b83d-704f-4283-9c6e-50036ca5e2ac','4a2ebf20-e694-4391-a3a0-4734c9928582','30d884dc-1d1e-40be-9f5a-7f159053f3fa','b8937ec0-340f-4c20-9c79-a7992b222be5','0e4d723a-a8b0-4656-ab28-e18716554577','cc840d7a-7dec-4a9c-9467-675e5ded2dfb','21f5bbcf-06d3-4562-b656-635c895e7415','d31e0c27-e4b0-4873-a080-378c9c7b5af8','9e7d54d7-b763-4189-91f5-f7d704b7ed24','9f3119c9-ca48-41a0-801f-21e8908e5f09','d7879ca3-9737-4556-bae9-c4c95854a391','b8bc3884-ed7e-4773-b228-23811383f9ae'}}),'106714',struct('BlockId','d5c866de-904b-4a76-82fb-63516acedf50','SignalIds',{{'435e4df5-ec20-42d0-82f0-7315465361c9','04b0819c-f490-454a-a622-e63076f40c5c','3312e866-e4e7-44f7-a201-134b32760526','9de3e8b2-fb86-46e1-abc0-f0bb4d28d0f2','02be94a3-ef6f-41ce-b8b3-205b6e8fddc4','e4672fd3-c283-4bac-a9e0-a34b760197f9','bd806596-9f95-4b5c-bed9-31e436472376','932eadbb-09ba-4212-a05a-551110cd59cf','1a0ff6d5-2bc1-43bc-9145-e06e20359f9b','f7526349-278a-44dc-86bb-bf6725644af4','078b2477-9f9c-4f2b-9b0d-32f32a1c8fb6','234cdc68-7568-4a76-9a2c-24bc86179f95','4374a053-62c6-4273-af08-a5f8072c059f','af32b2ff-8de7-422b-8936-b8390e86173b','e0a48eec-8ef6-4834-9cb0-37c5e6684c99','e59522c4-a879-4406-97e2-d8ea35dbc1cc','3a2e81ba-c9a0-405e-8900-da973159d78c','314446e8-e8f4-4334-b367-460396e58bbc','56133baf-ed02-4bf2-9ec4-cc6764fb0f26','a6c1849a-84ee-4dc4-802b-6aa411cc317c','97df8ec0-bd3c-4826-a4ab-a008b02518fd','4c754ce8-7002-4e77-aaad-344b79c409cb','88489552-3943-4628-90c6-5897ea18c311','45ee52fb-4d93-41cc-92c3-4e8ef9966219','32ebd8a6-c2e1-4d09-b505-4ceb368f4918','cf6860f9-d04f-43b9-b879-260184a5d41f','6d42546e-a794-4f86-adae-ec349a164d33','f5287581-4ad4-4642-8483-3210ead0b2b3','8b2ac739-9cc9-4cb3-ba6e-3bf5d384be50','4a64be52-bbb2-49ee-b263-2170a1968947','3d5cad5b-57bd-407c-9697-065d64ea2ed3','a422a971-25d0-4269-ba4a-e8b863ddcc80','84a774f6-6857-4b0a-96fe-34b8bfa68a24','c4062fa7-11b4-4797-96d8-cd0756ddd457','4be8a447-d962-4e89-96dc-13024a9d12fc','b82c6942-393e-41cf-ba02-c720dae7736b','94992935-b029-4308-be15-931fd9f7f326','56ce86ae-df97-4a4d-a528-df0ec3ced266','3794b3b2-f4ca-40e0-9243-9d72602485c3','e710917f-d59b-4b24-ab09-6c8d5fd685ee','b49aabc0-0abc-4e2f-93d1-31579a9f1655','22987836-8e88-4df6-9a28-b4451f9bd30d','211dc564-810b-4f85-8ca2-0afea1030e33','0e83fc34-07e1-414c-a6c9-e31ba0f52428','8ab44e63-bdc0-4745-9c89-1757dc52026e','fbe8e029-7d63-41ce-bb69-aaf7f11bebeb','0a012b4e-501f-4b07-a263-fd44f0e9de09','222ef8e7-84fb-49f2-b292-f568efbfae91','6736bb97-3249-4dcf-8b3c-cb75625b6345','fa19c8a3-88bd-4fa0-b478-7ff68e356df0','32b12f89-d5c7-4131-8d31-37c47ab1e691','16d9161d-df51-46ea-971d-60d5f20ec7a0','b222e43b-b6ea-4dc2-9e65-70760fc15ce7','548eefe5-b582-4c62-9a67-72b1cad93020','7e4fbf7d-54a8-4507-af78-97b69ef86a8d','dbbfcfab-7b98-410a-a468-12d6f62b8431','ee50d2da-21d8-4dc4-9787-f04791c1731b','536893e6-5258-4af5-adf8-380a7a48ca2d','5e030a7b-cbae-477c-9592-72c0a10d468a','d796fcb3-fd6a-419c-bebf-a3e250b89c74','a8bf7dc8-3656-44f1-82be-963152726375','de866299-d8b2-41b9-a010-f81046388f79','7ef601d1-0799-454f-9bdf-8e73025e4f14','a6d0c2af-8146-4059-af96-33270b82df54','17a91e41-f82f-4395-b756-21334dfaae8e','970767e3-7ad7-433b-afea-22257392bca4','b657a3bc-3db2-477b-b48d-252f29d713a9','1da0c6ff-24c3-472e-8460-cea4de52c753','b6b2bdad-3172-4f64-9fa0-c3119f1248cd','a656cec2-0d05-4d65-8695-43ba36e2f7be','dca7e427-e51e-4a34-af8d-e9f760aa608f','e1097016-c54c-4977-9f95-78cde8854a45','b7e20858-0a14-4ea5-ab12-584c7bd4ce01','2cc9b46e-fe4f-4fb2-9cf5-3933e3f18d77','5d888e46-01c9-448b-a772-fbd6072fc3b0','4f5bb553-78b5-409b-b7d5-04445fcac41d','c544b397-ee16-454c-b925-22fe831c6549','7549cd4f-3224-4c3f-a201-0e80d0403083','6a366e2d-14c3-45d7-b694-ffe0558b490c','2d497dea-8720-4661-b946-04776cefe1bb','a85eb96b-9c85-4f94-babf-520f2de789dc','9e230973-747a-4b65-83ca-1a92184d0c05','2b071b9d-0977-4b8c-ba51-caf25cc579fa','0a0ffe48-1cb5-4008-8260-72df0e83fd70','24b60833-a5f6-442c-94d2-5d6d9a62d4a8','70d0e0cb-3884-4ce1-b0c8-862bca342c18','ddb73777-b47f-4026-89f3-aca6c9722e37','80f82b2b-7adf-486f-806d-c6f23604ff36'}}),'106715',struct('BlockId','ae4ad3b6-4fff-4253-a532-102821617767','SignalIds',{{'87f119c9-19e7-42df-8b57-e17a988cbe85','c0cefc0b-efc5-4560-a062-0d4ec44ae225','f86f67eb-770b-473e-b7f1-76c77a777665','511c491a-9147-4bad-87ac-8c859f844780','b2e643c3-ff53-4dee-8c63-18a48bc15952','215f86cf-5ae0-42e3-986e-1632ce244a57','cb514ab3-49d5-4248-b032-cffc18d99185','bf1dac9d-a94a-4204-8567-f55a3ddb7dae','f34072f8-3539-4319-88c5-90f94f92f639','79ad7714-01e4-4038-bb2d-ddd421ff87e0','1d454c4b-41fa-4a93-b52c-9732f3943e82','c1556fe9-cd49-4d95-9be6-621227b1c4d1','368a972a-1b4d-4463-b226-2653f0f9e63d','c7e62745-8bdc-42d2-bf1f-919a59e4b311','f0843538-5633-4066-b340-4d7ad9a5989f','74743429-a197-4f02-945c-9380b454d27f','e7be925d-ce4e-4aef-9a4a-0912ed74ea7b','60bdd33d-3fdc-4ce4-9892-a602be91ea8d','178e8e01-c476-431f-a64c-ef8967ec77e8','6e9981b9-9ba9-43ce-9339-1d3be7040756','84a5edfa-f6d6-406c-9548-4c44f3666bb1','d82e0175-cf37-4dda-9f7c-f3f5dacd425a','3609ac1d-77bf-4371-b956-a1885783991d','8f3e2a29-8e38-4984-97fe-ab7ad3f03ff2','9a4f9fbd-39c8-492b-a5a0-4890e7d4c1c6','13f7d371-b70b-4879-bd9e-8a4b38c51758','8a283096-7178-43bb-9710-1a6c55753973','ff09ca65-abb2-456e-a787-9dc2a8292e9f','7870117e-a8a9-4118-9f0d-a9d0cfa10b93','cc4059a7-b422-4556-93c9-6a2a06a0e88a','c80d1fe2-8505-4c8d-8940-d82fe56bd29e','0e2c4ae0-b262-4d00-a2d1-55d69412a88f','6f2e4e39-a426-4844-bd55-36a1a063ff04','df1d30f2-c523-44c6-8898-e8d34ac8632e','61f19b5c-0260-4023-9eae-0ee4a4064b2b','7e974089-17c0-4443-9f48-f176357ca4fb','b7b85141-a332-4015-8d1f-27935395dbc7','4ceb984b-9f30-4afa-9d1b-5944c010b8d0','01b8f272-4f41-451b-bfd9-67cb30a9fc04','f51cc241-5a71-4daa-86ca-69c649a4a385','ed9e47fd-0198-4192-bb23-13de1025d7a2','22225987-5d5a-4760-be97-3f61b7a99804','2b6cf3cb-5bab-4cf8-b35d-8ef7241f1cb6','7a71a32c-17a3-4d1d-8f8e-85203f4c655e','42537425-b67a-4c6c-854f-115507550665','d555e7d9-d3c8-420c-b6e3-f346e88476dc','609c7608-9522-4826-b278-a6a5d2574f73','63d73d91-e8ac-4dcc-a8fd-af617ecdadbe','4d1c063a-44f1-44bc-be13-50024f1bb55d','262ca531-6dc3-4c1a-833e-7dbe2f459127','6f34e73f-45f4-4e69-b254-068ee5afcc46','bf75665f-f0fd-461d-ade6-4cd0059337dd','0da231c1-f9bf-42cd-852d-f778ab20fc6a','34c1d8a7-df24-4859-bed5-a0265c9b2b81','d39f73d0-7470-4234-afa0-b4afcab940d6','18f90840-7029-4068-9f80-fcd7175aceec','f4af81b2-9ea9-4278-b96c-5efc36a4aada','1d78e770-28f9-41f2-8b9c-4af23aab8025','693a13ee-12f2-42a2-b458-0bdf36499e4b','2a6a481d-df4a-4d5f-8284-dce8046d9894','91ccbae8-cfd0-46f2-84cf-21f00b6da56c','fa30976d-8ddb-49da-80f3-88a9152d6a76','1c8021df-4584-4ce6-9802-173d02dfa42a','87f8610a-8186-45f5-8f42-71a40e11c07f','8134fe54-e0cd-4800-b1cf-6f3697af4e0f','c28487f6-fb27-435f-883b-8df39ea0bc8d','a0005388-afb3-40c8-8082-e4cca5bfa46e','f953ca76-080e-493b-9a53-49b520d998b4'}}),'109003',struct('BlockId','0da86a69-dffe-4b7f-a283-8a9241d23c50','SignalIds',{{'5af6d936-27fa-4429-8879-41af435e11a1'}}),'109007',struct('BlockId','8a0e067f-6760-4119-9bf1-7de06ec4976c','SignalIds',{{'25c2c32b-acd6-45bf-ae45-1d49d7ac6f6c'}}),'109009',struct('BlockId','4622f2ee-7b48-47a3-9563-73ebc61dd29a','SignalIds',{{'c62c84cc-cbd7-47f1-ab55-08fb14620b34'}}),'109011',struct('BlockId','51b3ac0a-66ff-4a59-803a-cfe57852cf12','SignalIds',{{'b67f3651-4ae1-4318-a0de-88facef5121d'}}),'21535',struct('BlockId','2585067a-bea5-4000-9f4a-5d4a5318ba82','SignalIds',{{'61f4e782-3c5c-4d26-b38e-7ab3a332c17d'}}),'21547',struct('BlockId','85c6324c-04f2-4bb9-ae49-a2215b872cec','SignalIds',{{'0e3885c9-c264-45e6-aecd-762fe1b73c31','1baabd13-ee21-4652-b6d4-ec6abbd58849','7652d1e7-3cbe-41d8-a4c1-1dd8e2fc5cb9','7bbccffc-d9cf-471f-ab9a-2a8c4994da51','a802a3dd-5a68-49d5-873f-4e8d27fb760e'}}),'92418',struct('BlockId','c5a7be29-3173-4b9a-a890-b4cee331cb8b','SignalIds',{{'79a90cdf-8a9b-4ccd-8944-69c4469088c1','35cd3c97-8160-4258-a864-27af0ad45a59','a068c4ce-1004-4dff-b2ee-cba0a0b81dfe','05630d0b-4185-49b8-8feb-e160bf4c7342','87327782-42c8-4aa9-829d-57e10c6a236a','32ec414f-0201-452a-a464-db511b140477','a447bd14-b398-4e67-a61e-10660811da2c','bec63126-1009-4953-9712-db8f6ef516ed','b2eff86a-b6d9-46cc-97fb-d1becbbdd2bf','de8cb12d-21ee-4317-92df-23379c880453','5f05ca3a-8a5e-4853-a5b7-8c6c0dcf0e8a'}}),'92419',struct('BlockId','793c2d2a-ebd7-4dfb-b311-846f772c752c','SignalIds',{{'c2b3d6ee-be4b-4de3-95b2-89c4c1a90859','2f308f5b-558b-42d2-ab39-a19d3bc85296','12894442-8f81-49fb-bc96-47a5bf1bca4b'}}),'92905',struct('BlockId','c130785f-a926-4d18-80be-4f90a56fc66a','SignalIds',{{'eccbb9d3-c00a-4fed-9913-c35dfd825c91','c1e83077-f3f7-43b9-b95e-2f4abc61ed1f','b3378ad1-fa9d-4543-8cd3-a0383f142dc5','fa304a37-e84e-4267-8828-303f093fe0c7','3e860a56-b4be-44fc-83d9-afae1ad41a3e','c999cc34-3a38-46c4-8a1c-1fefdab530c3','fc5850c5-7bcd-4c27-8c6a-9a1a118edd15','71bedb22-8fce-41d1-b1d8-8abf9395d0fd','fcd7fb69-afec-4b69-b843-6566c7a71cf3','2f9a360a-3789-4020-a595-682571a650fc','7d4b0e51-2c7f-4ae3-b318-9737498e94cb','fc0bc73a-b230-4af1-a180-3ede73bf37d6','766856df-e6aa-4404-a2f9-666f11b78eb0','ab8c368d-5e20-4365-a424-76159427f1c0','cd802434-50ca-463f-b66f-d14e79cb60c4','efac5cdc-3a28-4136-adbd-30ddc781af6d','db1258f2-8f31-40f7-8b6e-1a61acd62137','765381b0-de7e-4511-8d11-c54a539c85ce','4e1fdffe-5de9-49fb-9c6b-b6115907f89a','d47039dc-7492-42a7-b7c6-a1ab58c33c7e','d4300b37-a6c6-4c57-a896-906157398140','331d091c-d097-400c-846b-e57d9b47c756','23db7ee8-2e7a-4648-ad47-b037c2972cef','7a92bfbd-8432-4cf3-bba9-5102f8da93a3','d6225bbb-9586-45b7-8ccb-407014cc48c5','23441fad-9abc-4183-87d7-b259083607ca','0dde033e-7c55-4e81-bed4-f372f31ef215','19299d9d-d888-43bb-8f47-8e7058fcb5c7','224da2ed-8488-4958-b851-20093da22004','7efba0e1-16bf-4181-8536-a48b5cd2d0a7','e73f4837-c9b1-4144-bea8-1520a76a6288','39f8688a-7822-41f5-ad84-d137df05f1ce','13253221-23c6-4520-91d4-b12ce5c98f82','2b2864b7-66bd-4bf9-81c4-a366357cca21','8c2ff0d7-259e-4a1d-bbdc-07d0c2fd0dce','9c98bbee-a96a-42fd-9207-e63e410c9150','ff62db54-7a7b-4950-95f1-e767ae3f0f49','aabaefa4-1632-40cc-9882-d40a0daaa608','5c5c25ae-9e86-4fcc-9c48-44bf11f46d67','75186855-9909-40bd-9e53-cd5155d778a7','b2114956-6d65-4bbb-9e37-67f3500147fe','09c2ba44-b82c-4619-9656-42a1607dfe92','af2f1598-0ea3-4de1-b7e3-52d79c962171','fd707be4-0fa6-4ae2-9f60-4370b6144153','4567b165-8011-4f30-8170-b653fb7ca9ca','ce1b30b2-f922-41e5-b8b4-db9281ad7f48','981d4ca1-9a18-479a-8eb7-d9972585790d','2c9ecb52-7d2d-4aeb-9d3e-a4c1e8b56aa3','95828839-e7d4-4a62-bb80-e66eb611e1d8','a184c7dc-5258-41a4-8c4a-c1be98591e3f','35ccfa30-c7db-4b04-8d9e-77ed7147eedc','eabdcf25-6724-49c7-8252-2b7db0dc0620','9c5887e0-8426-451e-b3ad-01e654ac3baf','1ae96621-426b-45df-b021-87aa2e52cd1d','89e9c9d5-36d4-435c-8975-5c50695f6420','c37a17f2-821b-4110-be36-51aac86393f8','7bc58ec0-bb40-4800-a223-2e444648b98e','e633a30d-f132-4524-b75e-0d9f6e9215c2','90ddf5d2-13e1-4ad1-961a-537e55784248','7d166e16-84ea-4099-8464-ce279385cc24','198a9685-b37d-47d1-909d-4bdbb172482f','2d281c1c-a91d-4a00-a1cf-9fb8696d6c2d','7872f9f1-7e80-4cb5-8ed7-ff8be80c0e6d','9ba31d8f-2dc0-4834-a390-6e97d705a4b7','107d086c-475e-4b0b-a20b-5263a4427ef4','c3d66b39-b3fa-4845-b3f3-5e96d6860841','49e18595-2bd6-4e15-bc14-e9bb0458c226','2f88091c-fe89-4fe7-a6b0-adb380293617','bfe86deb-ef77-4a46-bc27-242d234016ae','72347ea7-d7cb-4ce7-afa8-b3b4972bf273','185e8e44-603f-44a3-b375-4ee1d80c6d3c','e6479db4-b6ff-4f92-bfaf-5af0158b2bb2','4e72e28c-3ac1-4177-98cf-6ac5a77a5b5e','d3e5cb8f-1aee-4ee7-ab68-88242de410af','d6ccaa71-6906-42ef-b48f-158ba10375bc','fd28349d-425f-4f21-84e4-1e9d232cfd82','a8d07bdc-79da-48dd-95f5-7ed7f0ef04ca','55b165cd-91b4-4efe-b4ec-5ce94f7b842b','65d838a5-3c8a-49f8-8107-95e629dfb205','36d6d967-3880-4484-8ff4-a86fe1881e48','f6c72526-ce4d-495b-be35-b87b229b2ba2','eec45291-cc04-4e1c-a4ab-647c5bfd71c1','4b49273e-9e1b-4ae5-ba38-9efe2ac32757','a557b5bc-8dce-4849-bdb6-0dfbd7ad1634','f827e4a0-73ed-4c19-a1ff-1dadc01fa3c2','e01418a3-d7eb-448d-8a1d-9c482990fb45','fd53835f-8adc-4332-9675-9225dde50eee','c88b335f-0edb-4359-9f0e-ed3e41c135a9','1ca6aeef-ca86-4006-8e7f-9c30a846fa44','d1241a90-d6be-41cf-bc3a-0e70d3e7753f','0e8141fb-7cf1-4b72-a43e-e22f9a0bb087','431e77e4-059c-4159-9827-995b426ef671','b8191d9f-f149-4649-88fa-da5c454439e6','994e95d2-7243-4545-bee4-be9dc5a78f58','25192014-8c94-4646-b348-bc138f289d24','5e84b834-0fb4-4ad4-8fcd-2a2dce8d913f','1a356363-9f26-4958-b4a1-5e3a6e32d08f','3b5b7448-3497-48f7-9869-7e4b9c495140','1035105e-2e8a-495c-863d-a1eeb2b28d38','71e9e0c5-50c3-41d0-bc33-6b197c083dc1','dadd1dae-354a-4e35-8af5-93c2733b6673','b5f6c23c-d3e0-41ae-968c-c3bbee34b738','9167b3aa-d85b-4ad5-af82-aa511d6e13c1','a2429ab4-7fb6-466e-95f1-25f4313f44ac','4dccfdf1-f6a0-470b-a153-ffa6f648f821','91fac8e9-1560-40cf-8ace-1c69d952fb6a','db9d0dcd-a444-4f1e-8b2e-60a63a3374d1','3ac30f11-b1a0-48c1-9616-3a84bfdc4541','d4dcacb0-037e-4ebe-8662-550bd9bab09f','2dd478a0-c250-4c36-a6d7-0f02170edd93','23d62cde-720e-45a0-80dc-ece62fe8a79b','6e695378-4272-474e-843c-bd0dafadb5fb','30ce05f2-a117-422b-9db1-53b49d33f003','c1eb53f6-e8ec-461b-930b-50d0fc08fafb','9302bf8b-8e55-4adc-987b-07bfcb9545d8','c7607c18-f485-49c1-bead-7614f7675b80','462b230d-e73a-47f8-8636-a327ffd7af4e','c2ae1a38-3545-47d2-a39b-48b2b8846a32','309e70ca-9895-4830-831e-7b47189fc5ad','0ed28340-889f-41a3-8b47-96d565c82289','e40fe7b3-99dd-492c-9823-52ef80d6430d','247fb40d-f9fb-4c81-a48c-da761156d76d','128fd641-051d-417b-9ce6-5eca029ea2d1','6e9100fe-c71d-48f7-bde7-13fd4d174316','a763e0d3-aa72-4413-88cd-b58f59d1d542','5cd57557-0a7f-464c-a737-3e574a22fcdc','2d740061-e092-43c5-9b15-f853d25f1ec5','54bd9f7d-823a-4bb1-ab37-c593fa42ed61','76fb97ed-a42b-473c-a1fc-027e2468af2c','ced7ac28-2e6a-4465-8a9e-625670ab4739','55323f97-af53-4383-b6a2-0bb134c7a4e8','45090804-d81e-4ae3-8646-7e8605c13b7f','c9c75103-0220-4a59-8096-57ade6a91c03','25d86eec-ee3b-4683-938c-1a51e105ff89','8b609c77-7dba-4987-9c70-6b40126ba1e5','4b8ababf-d535-449b-8eaa-916cb4c74271','ea6cc9b8-3522-4aa0-9877-bd5b63d92e91','3b26b576-4814-461b-981e-b98f479dab53','aba15bcc-b237-40ae-84dd-255a4e5df669','32777c41-daca-4aba-b907-e608bce7966a','d64cfbfb-7366-4bee-8772-fa34de82d4bc','58a8bc67-bfb5-4983-b19f-5b22088a9dc5','f7f499d6-7f6c-4e69-95ca-d71fdf112412','1bcdeff3-6bb2-408e-b0b4-9cce5e3e5ebe','601db135-1a71-4ffb-b0f3-e0d2c7303cb7','fc4bdd76-7e7f-4d3b-918c-bedc9a1a4e51','93bb42cb-6cf9-495f-954c-90184c1bec26','7d92d163-160b-45fa-9ea7-a5d3e53c6eb4','fe38bc4f-3aec-43f0-a4b8-29da51bb3d3f','ba148611-7928-4b2b-a591-9191cbb0b363','cda993b2-d3a4-4bc3-a3d3-94734fdc5eac','0df8d57f-0157-4ae0-885a-9c7f57834c5e','805df1ac-18fc-40a5-9a12-6756f51fcf2d','c754ede8-c7e7-4b47-88cb-4cecd064fb34','080ad2b0-4364-4052-a15b-07bd221f6abf','c7e86b97-4987-4936-94e4-81fc0312c5c6','ce78cb29-501d-49b1-8414-f6251498dca3','8a1542df-a2b5-43fd-ac36-c2e6cf84a1a8','605d94a4-29f8-4da9-aced-83a6bbdd3713','1064be33-f0dc-45f4-80bd-05b861b1e9ab','354b98b6-3804-4dd4-83b6-64235718ac83','00b8994e-754f-41a8-bdcc-d7613a88bc0c','1d1c9eee-b84e-476f-afed-5bf4ca124a65','0eee1f82-45e8-4e06-9be7-8c9beed7d0bc','c69061c4-a914-4e6b-b48d-8bed2e9a00ac','6651c467-a2c4-4ffc-9b8f-28e699227aa6','defa2c95-1ac7-4863-b494-86589ab39378','fe409676-facc-4e39-a0ef-6ebee6abaa60','705f6a46-e19e-412e-8bdf-bebcd1b67aa3','8b693a7e-de63-472d-b571-bd6c3df47c96','40cbb4fe-43fc-438f-9ae1-58318ff1a440','a622d429-db00-4925-99b5-5a62d39ed440','e1e27195-a0da-4626-8332-95882467547a','b940a082-1efb-4ec9-bde3-4dd851a96c00','ab25bc12-04d1-4d6c-a724-a2e53496de1b','9c9570db-78f9-491e-898c-2a4fb64a5433','ba8a12c1-0bf1-4c79-af0e-64353e650818','ed6acb4e-be58-4536-9522-3d897eb19ec4','4c055b33-966b-4bcf-8fea-c537219c43df','e328c68c-36f8-4518-88b1-b91e692a8432','3bc9fe64-82de-43c9-866a-14697d27101e','69a03dfb-4b97-495a-9e48-ab6cf5ef6ad5'}}),'92921',struct('BlockId','01f22f4b-6e24-4088-a5f1-2f36f2b9e2d3','SignalIds',{{'53ca05e3-9731-4f4a-8cdd-0f1937e4e7e9','9f9e8808-7f98-4a4b-bf14-9a7145728ce6','f54ae71f-9e8b-4b6c-8eea-9983ededdb22','2fd0085a-b7d0-4ec4-9e7f-36db35712486','1d7b09f8-1e81-40bf-a417-dd63c4998356','78b3f90c-de19-450b-9caa-4f8c8c164b1c','3608bdb8-911c-4ab3-9a9d-37769e1dde4a','fd166d4a-241e-4f74-913a-30a8b0fa4015','e0cf4520-9965-475d-b149-4aa5db4c721a','b30fb91b-d056-40c3-b335-d9c0fd56e001','6a5f827d-2ff5-431c-bd12-921c7afc1b21','fee74444-d8e8-45ec-b62a-5fed8bca4dd3','89d91d18-cb6d-45a5-bd38-163652f833a5','324211fc-f604-494a-bbf8-51e05583da4c','9e22aa07-a035-49fe-92a9-2c6d331da650','37ac9124-bad1-4f96-859a-3d7c4c2d26d7','276947aa-f54c-4f37-bb98-1f5926d03c2f','56e619e1-414b-4fcf-9dde-3fa79bcae4f0','946ef8bd-4767-46de-a87f-4cbd09323be9','d2043996-b496-480a-ab8a-78a7b4ac0cf4','27abb0f0-4523-4786-8486-6e82d9c24a60','5a662e81-82ff-4260-a25a-ab47e0151bb2','543cc627-7fd0-4544-a7ee-951a14aeed15','fe10dc10-882d-424c-9725-783731f5e974','25a215e3-1ac4-4d7b-a2a9-86b28d91bb89','2bf23347-477f-4f1e-a5d6-520b47f0bab3','db462e6c-768c-42f0-a44c-89f649570b02','366cca5b-5193-49e6-9376-169206ac9353','fe81c863-cb9f-4014-b168-a96d9ea111dc','c06798d7-c97f-4175-a44a-cfc61221cf4f','36e41669-6ab9-4757-9a49-4ad9030b78e1','6ae2d8e3-ae24-4f66-895e-50156a7f00a0','7ca11891-0d72-484e-a2bd-2a22e9dd0486','4f0179c6-c3f4-4108-a3d4-fcd8c59b8d68','3317a0c1-8eb3-4564-b3e5-2a1f67eb9ce6','acd8a3a2-5082-476a-a057-e8342edfea73','0f99ac7f-474b-4f93-9e2a-18d8d6e0a2f7','ed037e56-e86a-4cb5-b0dd-1afd7d0cdc0b','e51c4e5d-52b9-4ba3-858d-8ccb1ed7b833','b102886b-794e-4f9e-8d82-cf9a855382d8','9ac2a337-debf-4080-8557-b89f9504fc31'}}),'95726',struct('BlockId','ef0b5d28-b6d4-4eaf-949d-d6dedf719559','SignalIds',{{'ee15b610-82c6-43bf-9a8c-0e7a9659ccea','3b41ead2-8f03-45d4-b3a2-152baba76f1c','04424910-0e7e-4b8a-bfb7-18efea10e449','d3e92efb-eafc-4308-a397-493fc39ce811','878e6af1-c668-4ab0-8e4c-5c6032b55278'}}),'95727',struct('BlockId','b2b56e4c-9e5c-48f2-8bbe-9899bbf5491a','SignalIds',{{'4e2474d8-d594-488d-9a95-ac26de9b628b'}}),'97162',struct('BlockId','609081e0-941c-41af-a124-0ef5d7529c4e','SignalIds',{{'7a0f8b5e-91b5-4be5-aa3e-8b6fa3ad27d1','46832e0a-dcde-4f52-aad9-ee2d5b2f815f','bfa458bb-0f77-4e22-9fd1-ceaff99b329a','ac728005-1b3c-4171-959f-ae8eff693e6b','008a89bc-e3d6-404d-8ad8-0ede00b346c6','21c71be8-3a66-4a2c-95b9-571df8448d55','201d8bfd-af86-4d0a-bcf2-2be355973df6','17b8c076-2f41-4633-b3f4-ebc4292cdb2d','ab00a850-8ce7-4b74-9f89-de7c76bd9fd2','240f9350-204b-43d3-8912-096b8d4fb3f9','cb628a66-37e2-44dc-ae8d-af5a0f7c0f4a','6af2e867-4ffc-447d-ba29-ba8626120048','9fcbe341-bbba-4ceb-b6e8-1ea49d1f1c20','a24cecca-e5e9-47ca-8406-22f227da4bb4','664c1055-c028-4f6c-a847-16dc729d939b','94775a18-8b75-4854-8d5a-a4dd0e581b4a','232f361b-601e-4443-b8a3-d4bc6ac96435','1fe87f67-5efa-4bdd-9d59-3c81b1c88557','81f862d0-8470-4c56-9e69-bc32aa30d43b','e1a68ded-277f-4555-a456-1524c13163e5','eab70a40-031e-4639-a10d-e5d41cb3f774','f526a80f-9956-4640-ab3a-89d2045f0162','edbb942e-05fc-4847-8de1-9a53f76b57c3','fa5191a1-3a1e-4763-8ee5-164c10c89699','50910d49-eab0-43e8-a422-548b52d3ac7c','0663fc9f-f5a9-4bfb-ae5e-87e83d32350b','eee09491-0338-41a4-874f-f2316d53c699','6f8a9a16-516f-452f-b2c6-592de3d56c59','d4fab639-aa70-4ab6-9a17-13486f62d987','8d916867-5d55-43ca-9700-dd7feeb9bc6e','eeb9a4a4-84f7-47c1-9ce7-0ef2f39b74ee','730cd9b7-4ed1-47c8-abb4-845d6e05153b','3a8d6f03-c7e0-4aec-b7ea-561ca6594a58','25840a63-a918-49a5-a812-8a1a8028e971','aef27282-f49b-416e-827e-cdd345ba9667','24938d64-a0e0-4af1-a018-252efc3ebd59','e37b8316-1f35-4643-89ab-21172ceb4edf','b22000d8-6743-4f74-a74f-a3205d460f56','071f6833-b20c-4d46-b3e4-10e823412cbb','ec3e142e-8960-4688-a09d-a55ea4e32adc','ad9531d8-6532-493d-beff-fe127dba79c1','d835263a-ecfa-4975-9fdb-449f341a58cb','eef83801-769d-4b17-8c33-06ecd7e9531f','5d0189f2-7d3e-4f08-8fe0-161cf62f662c','d2f707ad-9b49-432d-acdc-bfb37fb60912','1a39fb43-09e9-4f77-8799-5ac95783bd7a','c7276a0a-abe3-464f-bf0f-2f48a797c1e4','bd5870c5-724f-4d37-8fd7-060d6b5b46de','d639d805-c587-4e89-b332-581ad6e75f23','6efa384c-85a9-4595-b0be-cf78e9440493','53d8dcd7-0a8b-41a1-a4d7-7828db180377','9e7caebc-7806-4f8f-b588-3fafd79f3b79','2e9b888e-502d-4f3f-9192-523b6326006c','12683d1d-dbf1-47f0-883d-2f89e9585a50','0247e252-86ee-4c9b-924e-349beb4cec5d','dc694a7e-2623-4887-bd95-05da09f2976d','ebdd29c2-8c6b-4b33-8057-4a6975ea33fe','858e3f46-3ea8-485c-b4ce-1dbd84f5f4b5','bd26857f-1a73-40c8-81ea-009552807393','a67ed66b-0df4-4077-bdec-79f7b0742a37','41ba233e-5517-4492-8c6f-88d14ae87849','e89fef81-5e13-4cdd-8565-e3a4bc554c6a','79d59ed1-5a59-4091-a0a9-961027512cb9','3157c6c1-20b0-4cae-80e5-07c8fe13cb5a','96edf60c-decf-4636-b100-d32d9156fdc0','0186c05c-0b8a-45e7-acad-09290f940f36','8d0919bc-d469-4ad3-8876-2215fa1e3c58','94796f50-aca0-481f-b09f-bcd3b61dacf6','0211f4a6-eb10-4ff2-9ded-efe2f54bbcba','3fc8fd11-180d-4279-a4d1-d315f519dde3','95a29aa1-566b-46d4-92af-bb59b0582c30','74c5ffe1-f404-42ea-bd01-db28b37aef92','7582e1a1-8611-4d3c-b4a0-d1ba90126ba8','a38867d5-0379-4628-b738-91d324b276cb','1aeab194-b8fa-40b5-9dd6-7e24b15055ed','e65d4b7f-5403-4cfc-8754-8de4db2dfc3b','ceafec07-8674-4c62-89be-392175838a4f','571a7066-71e3-419d-b801-ed3605b6a94d','a339d5bc-4bac-4202-9add-1e8b4b128418','38834dd4-1316-404a-b5fb-2b6d10676a60','28b836e1-ae50-43fc-84d6-d9ce7b6871d9','7e48a4f9-6a73-4625-9ca2-29b40c8ff1d9','a2bc4953-5b0e-4e1f-b774-6d10007aa0a6','f286eacb-0890-4462-b3f9-5db0fafdecf3','86954f5f-41ea-4f72-bccd-7539044883f7','da475526-0c4c-47fd-9fc8-9468cf6b7138','eaf5dcf1-085a-4450-95d8-e0e1b31b251b','8df4d6d9-a5f5-4230-9551-006ec052d287','a6905aa2-b44b-4297-9a6d-b056c9f0f561','7c2775f6-bb4c-43c9-a1c8-611712bdfe50','f8aac724-2f6b-4507-96c6-fe2b499ca7af','c6c5d193-f81c-4525-a928-e534762a4996','1b3b3208-9784-425a-91f4-316eb01c5c0e','120ab8db-7f87-4a6d-80f3-9796dc49379f','6d4e0623-c660-4980-bc46-d841b5f15fbd','196c7c87-e6e8-439d-9c9e-2d0be2a1badc','914fd7ff-ce5e-454f-a0dc-6be5016f04e5','8fef58bc-aa80-45b7-99ac-679676dedd7e','dc22e312-d229-40ff-8255-43c4024e57f2','ea3a9df2-9771-44f4-bd80-87ab18d08c8f','d45e7130-805a-4cda-94b6-fcfd560accf8','332ff65e-4f46-4811-9c0c-aa49297458b8'}}),'97187',struct('BlockId','28a1268d-6eb1-4b71-b208-78f973de8d60','SignalIds',{{'585913a2-9f2a-482f-a871-6411ccfb653d'}}),'97198',struct('BlockId','d5a98707-e9c4-4286-94a2-1770c80d7f4f','SignalIds',{{'c855aa43-135d-4843-9f79-db840653e8fd','54417ce3-4c9d-44b2-a33a-25590b836b81','47cdef3c-44d5-42c9-abab-8063e32dbde2','c6425e0d-8cb7-4b97-9fbe-624d35a3e47c','77d2dc99-15fb-4ca0-8459-b10db5f54984','b06d46da-0afe-4348-9620-4a48ae4589bd','99f6435f-1975-4fbd-bd5f-98da826c52d2','e20ae6f0-ed78-4f04-81af-c59b4fe103ab','bb3ddaaf-07fc-4bde-931b-8b2831ae140f','369e9b5a-187f-4111-aa6d-64fcaeeff6b6','0600b854-4b29-4c2c-b5c2-771f8ef656ef','3d8d12ec-590a-4d9a-88fa-80749b59276c','a3bfa13b-5373-4658-bc35-8787c30741b4','b6e39718-75c0-406a-a8f9-b4ed2f932d63','3ae9b18c-9a42-4f93-bd17-c5884e555cba','4407ef51-ef66-4e3f-8e23-bf2f84b36441','80162738-9f36-41d3-bbbc-cd6f71812cfb','145ed585-4889-4f43-a872-6ebb3f7d528f','14ea400c-c0bd-4096-a660-ed8b908b94a1','e52b016b-0789-4cda-8e41-4c5419829fcc','d084e8ea-b9fd-47a7-a81b-404462515d73','14127863-cd8a-4aa2-ae63-f72ff16a2976','4d6dd348-42d5-4e2f-9857-af5495f942fc','9e1ffb98-cd10-47c7-bfa0-c7f82980d00f','ee3cfac1-8666-4d88-af2f-dae314b9dab0','32809660-4ebf-40a4-8fac-00ba1a8694bf','9df86f16-1321-405e-9e8f-6b65c0a77fa6','bd514d21-f259-4ce2-a044-75cb8241019b','4846c61f-afc7-4cd4-9014-9664af955811','386dabd0-67fa-4157-877a-5d180a615039','49f7453b-7d25-4dfc-a6e3-96b47f9572de','b88020d8-7bff-4d0e-bdbf-e55a3db9d2bf','f1b13c7c-ecc6-411d-82d9-5440c55df978','13a9fac6-3b2e-4e20-bb2d-49a8badf1a80','26f9ad9c-eaa6-4a90-a5c3-39f447a9ac78','0af830f9-f5e6-454f-91de-cd60639fa1e7','0560ab11-f83f-45da-9f12-4a6919fd4ced','29d2492e-438e-48be-9926-d533d6feb313','872e73e5-2920-470b-9957-414be0968712','e5f43741-853f-41ce-8e42-68a48f704f7a','43f3f7f5-28a7-4c90-a4f2-0b63d3a25f7d','a968688d-5a25-4c23-a524-134b79f7ae05','675b099e-8b6a-41f9-b872-a4bbd499150b','2ef6222d-d808-4404-8286-93450e58a407','6d426830-ae0e-4b9d-8b8e-c7a48734a28b','9d5335f9-6bfb-4110-bc63-fbe87897593b','b9f0f5a5-b551-4e47-927a-8ede67aa92d5','9afcb1de-463d-4956-bd81-daaadeee848f','22d4c151-a8b7-4096-be9d-b0fdf8528350','edfca5ed-cefb-4e7a-b682-09011c6dd0a2','27e13cb0-125d-429b-bbfa-79cf555714a8','b14b42fc-9505-403b-91f6-3fc60f9419f1','f11f7922-4891-4d2c-b4eb-aab8199e3756','1a5d8126-688f-4f87-92ea-4dfc2f81fe73','07a9e82a-eb3f-4b00-8031-1d46832aaf29','fda4505e-cb50-48ca-bcfe-4ac1460b16e2','3b2e4117-90d3-4408-94cc-bf1633040885','b0df4232-7da3-42ab-9f51-717797e8d978','89c96393-e15a-4f8c-a0bb-5addec976af0','ce89c7d6-af94-4858-9886-ba85618ff3d0','97b14e89-7e16-45b0-abcf-7b63079a139d','2959c2fd-b9c4-43c8-ae3c-0bf737823b3d','7b7f07f8-d0af-4756-8660-6fcbc2323be3','44f08197-78c1-4d08-b16b-972ccb00d32c','47ccc443-dbc0-4163-b94e-3023e1cc90f1','fee7ad07-4aad-4075-899a-d709b7f73b9f','b80ed905-e196-4089-9d38-a63c4fc3e0ff','eb35c15b-9175-47d7-a1f2-71b557a9f887','6ee26301-5de0-4a4c-876e-bac75a633ad9','e386771c-ac00-4ed2-a2fd-067c02672470','37b5cf25-dfb5-4e8f-8246-fceff19a7fd3','2b936f37-24dc-43ac-84d4-c56aa3fe720e','3931ff07-50bc-4616-823f-daba0e6bf238','3ed67b90-0b05-4a41-804c-27b0d840a85c','c1b8f6b0-29a9-4807-9733-a3d0e1039b03','067383c7-cf9d-42c8-a878-9e46b76d93a9','71f564a2-ab04-47b7-8890-1fd2a41ba090','8314a54e-ae40-44d8-bd1e-e3d36f768aa9','ba08720f-0ff3-454a-a0d8-77c8e3624210','65821741-3b91-4356-ae05-456002bb6637','013b88d3-b79b-4d63-a4ba-78498664be62','11e467c6-4f8f-40a1-bb47-6f5534593064','86b552e3-fb0d-42e3-ada8-6fb503052d11','306eb17a-03b2-4afe-8c47-fa019acc3e5b','5f9aacc0-8a99-400c-8122-8554c024806a','1c4ec95f-4377-4e8d-81c8-17e0409e5374','d5f1f4b0-a4ec-4d78-9136-f7381469164d','1932bda8-ec34-4aeb-8f11-f5cdfad08262','ce1a3840-3719-44c6-a444-2d6cf192911e','c028750a-bb52-4abf-932d-7b5a6a5342d9','87183d5b-ae04-4daf-85e4-c88dec1a53fd','8009f076-f77f-41fe-9ff8-e2e1c0c42177','5940b7e9-f37d-4acc-ac5a-f3f10831f659','1561e29a-0bae-47e8-bccd-698a30165295','74a6ff88-a32f-4536-99a7-5c33638ce392','afdefe1a-e3a3-42d4-8967-c18a8b333b14','241b2513-728f-477b-8232-42d66631417b','28b79b5a-055a-4112-bd05-df066b9a7adf','fc21657c-150a-4547-8e02-1f2f56db70b4','9574e010-78dd-4311-a59e-625492259326','b264e420-53d2-42f7-bc0a-3d486e1f3dcf','b1a0c23e-c8e3-4cf7-9b86-eac31ff31471'}}),'97223',struct('BlockId','2bb0817e-a54b-4064-8246-157ce30e8a45','SignalIds',{{'7c35180c-1def-4620-8cfc-ba0748efa5e5'}}),'97304',struct('BlockId','4118e63b-9826-405a-808d-6a2815e4502d','SignalIds',{{'01b3e1a7-f378-401f-8832-c17bbb23d801','8bb1a5ae-2220-4e72-911e-1bf42e58e4cb','dc537a66-3ee7-4b74-a769-466a6749f5f3','cc345bca-7163-4f98-8c36-d8b285b2316f','72bbf11b-86b8-413d-a3c6-b15ad8f593fa','09d8c20e-ec8b-4845-87b9-7498aee8976b','6f95cbe8-f55d-4f50-9a94-a1486b31b339','e42558b7-a07a-4146-9aaf-d538d4bcc547','a567dfdb-8fcf-4ff9-a1d2-e4b8ea8e87b0','a4a04237-9ad9-472b-9cc0-cba6eccda89e','d21b2fec-157e-4546-99aa-20a49f5b2123','cf30603d-a017-4758-b4ef-acc10542d365','f97d1c5c-89fc-42d1-b443-04b1f4566020','e5ae5f93-2521-445d-a42f-5357582259bf','1b59a933-7082-4e42-b5fb-636e4d03095e','2f90ca23-1adb-46b2-86d7-31ad12da6482','0f36c745-20f7-4ef9-9082-da06e169bfa1','061d2dc9-9131-4b99-b48a-9b0ff8d8b97c','28be56c8-312f-4e5d-b18e-1edfd44a6e2d','0e79623d-4bcf-4cbc-8070-38f639d67d18','908c7efd-3bd6-4f85-a3b6-9d52056e9c78','1cca5fa1-9e04-4d62-9101-d6ee7080ce3e','a775926e-0f86-4205-af19-7b70071a253d','19793d7c-79d9-44b8-b460-0f82d260e67f','9ca958bc-1b2b-4afc-b1ae-7d8be721e757','93e3fff1-70a8-4a0d-9417-b9de293bd010','ba446519-3a3b-49ac-89b8-b12cdaca3106','b73d54a4-a414-4181-944e-1eb485d8283c','89d5975a-ae08-413c-887f-694367b6d4b7','3175ec4d-6a41-4088-a19c-d2366275cf89','03dd4b3b-b690-4de4-8e85-f63146e35258','60627bdd-944c-4e63-8d05-4ea0006561b9','7cfda0de-925d-402d-9482-3f6fb5c606f2','240cbb01-d769-4a55-9c48-191c9f95868d','6832e2d2-1db0-4b5b-acef-28d647aab0f2','677c103b-6c9f-4bdb-bfc7-6fa9b6622754','cae61037-28de-4d53-8c0c-8a4e07abc496','1e5e87e4-d961-4212-b768-b5a8cdee5839','d5531e03-5688-4968-aa6f-7cc3599e3350','92e24c3d-ceb9-4877-95bb-ac81a5f8d155','6a1b7d30-ea42-4d8f-b0ec-1e21fc93c1cc','4559e5c9-5dc5-4cfe-b9b4-35e2b3daf863','c80a97dd-3775-4c55-94e6-856feacce23c','1f4b3783-ec57-48d5-bda0-a9f90bd3245e','9163066f-f49a-42a1-9a3d-15ea6dfa20f7','b291e216-46de-48e3-bdce-9d5f83f81ce6','7d72d178-26c6-464b-baa5-cdcc786b292a','b93ddeeb-1b31-48e9-b7ef-934d2a9e5c49','ab219c3c-0350-4a60-97ea-db06c4fee33e','6e3b383b-48b4-49c5-8c97-d9f877d2d3cc','7b66c355-0d89-468d-896b-3bb056f5e6b0','3b02ee0a-f6e7-4055-8a74-f81765a62fa6','98edbac0-0bc0-4275-b67e-d83d083685de','f12b0a52-09d5-4ab5-95d4-376bf9cdb91f','58e7d122-3c14-4ec9-be76-5a19bed4fc74','545ced7a-c299-4d81-a823-688beb87c278','8eb9c465-bca1-4103-bc99-d8a256cc79de','13a7d792-0e73-4cb9-8b76-7c831f116066','505c70cf-0ebc-4438-af82-c82737fb82b1','36cd3976-7cae-46c2-bc66-0783780c46f4','44ad4cb4-78fc-4870-a22a-c5737ca7506e','0f308031-0ae5-47ed-a451-2b0a8e74e6f2','69f4f3f7-67b9-42dc-bc25-a8b39ba3090d','080e6084-e7a7-4dd4-8b1c-1c43e9dcd6ba','74a9494f-9873-4c2c-ae76-8a0f74db06d3','ccfa1334-ed0a-46c5-b27b-0d24b3fe104c','02647cfd-7651-4591-82c0-c306a45d9954','bf5909b8-e47a-488a-97ac-8a8bb4162d68','1b52b0ef-86a9-4dcb-8cfe-32aac3b81ff3','3598f962-26f7-411e-8435-40818213f22b','1e0211c5-e0e3-470b-b0ee-33e8bcc4d108','5c746092-0c30-4e69-b43c-c92dfadd0b45','d778509b-398e-4732-8971-0ff5cebf9cf4','04576cc4-8882-4415-afa3-aeedc508a3be','c024dd67-34b1-45e3-a631-5b7bbf918376','11631a09-793b-4867-be22-79d9d65612c5','a3357929-da2a-43be-aedf-f6305debcea6','de752852-aa1c-48f2-8ef2-374d2db6bf7f','b12e6e17-85ea-4152-b69d-d16c6eb749a6','374358cb-0fa7-4c8e-92e9-037c0bb44a3c','1804bd15-cbb0-4ab3-beb3-6ef8ee465187','91472f63-d464-4e24-b37e-63823e391a72','373b3a93-b019-47b7-baeb-06c0a5a55f6c','814253fb-3bd6-4d1a-a9a5-a3f852134056','3b484bf5-91e1-4a0d-a7fa-cc4fb327c5c5','ab27b948-cf6e-4c05-947d-dfb2c65438d1','2f1b953e-1e5e-4065-9a7d-c6a7bad72005','a9f5e343-41f1-47a8-9445-7de5b8319862','0b7abe1e-ae09-4c9b-b38f-26afcca63e63','120ec359-a99a-45a5-8978-ec6ad16a0a24','a1386bd1-b3cd-4f88-82fa-66a9c6dc047d','27ff8947-825f-4a8d-b1c9-e78d91e1fc65','e484b846-ac39-427a-9333-a5dd0679e88a','a023f569-8a9b-422d-8e35-98d8b20c49a0','c6fde034-a3b0-4ecb-bb08-4786cdc61482','1ff15978-77f0-4230-8db7-739deffe4e18','2dc576c2-15f5-4b47-9974-0fc4caecf4ae','3c460159-3a51-4504-a157-b91f565eb795','5d8de635-6c66-4c6f-a0e5-69443bd37ffc','9f232409-b5b7-42be-b408-d2f2a0fdf988','0d56aaad-3931-43d6-9944-cd7d8d94e774','7ae3225f-bf53-445a-8835-56fb9d6975de'}}),'97309',struct('BlockId','c5b8f01c-70df-4224-b497-d544796a9d10','SignalIds',{{'42317a15-fedb-4030-9b34-a5b724ca26dd'}}),'97340',struct('BlockId','8b0a5312-a67c-48a9-b34f-1d6be82c8843','SignalIds',{{'f4db5faf-fb61-4c6f-b640-80cc192d1c8e','0a8a547f-22d8-4376-a9b2-5714083fb1f0','1208775c-8773-472a-bbc7-698634299448','ca05a6e5-cf91-4f1d-bc4d-28b1eef3c49d','d8eea1a8-aa7a-4d6b-8051-6bd9b610858c','5c7a2e4f-ace6-4026-a188-f979e1be3eec','bdfdada9-9c4c-477f-911c-c65d9e1ff339','2a208145-772f-47ee-9a7b-1aac75928245','0241cae5-c55a-4a65-bb99-da8f2c93baa4','4eb98ae0-8f8d-460c-87e0-ed84f1337715','a415dc3f-993e-4c04-8f62-408ce761464b','9ea75a97-370b-4a3b-9631-8371a94bc6e1','bab598bf-ac29-4c30-89d8-a221a5aa8c31','1aa88398-2c2d-4566-91b1-886bf2739ca2','435cceb2-096f-461a-97e2-2803eba8e13b','bfe550e3-05f8-43e0-92e9-29a659165fe0','575066b2-5f9d-4f7a-aafe-06d054514401','1708d4a7-b108-4092-a880-4a9233a5db3e','73bfa96d-f7ac-49ea-ae1e-07195bde5abb','74affeca-f459-4b5f-86d0-0c77c6a80cbb','bc634706-744e-481b-b24b-00ee508eb29b','740ee232-137b-42f6-a63b-d6fc7bc48afd','12569f31-0a11-4715-ae9a-329e667c8980','e6c015f0-2974-4f95-a10c-da91412374fd','4387b9aa-8d23-4a34-abe7-732fb690422b','053a1b06-d267-4261-ab75-6cddd42f835a','7ec7c7a3-3230-4240-8e12-f8259b3e50f5','4e427f28-e16d-409f-8c34-1cf947def933','4334d358-33b7-41ad-b6c7-bbbe6a15cd96','641298f3-8099-4649-a67d-48c86f0109c3','fece37c9-e9c1-41bc-9561-ca5167e3760b','c3eb5f33-0244-41d6-b000-ef71fdcec568','0423900d-d6a2-47b1-a914-20055e321f8b','2a8324e7-3ea8-48b0-92e5-d055fbeb7eab','6642d8fc-9171-4ea0-b94c-c96c126fc14d','3576bc2a-e5e0-49ad-81cc-7ebab95dd16d','d2b19811-e4b0-41bb-8d49-39b3e6b99fb0','915508e0-5c5d-44f1-9d3d-642b8c880c17','d8b08ebe-0925-4d0b-87db-03c30dda66b9','f4818373-bf5d-4163-89c7-b21ae55be742','96242654-5563-4c8e-b566-d07fbfac1306','23f357d1-3449-47e0-94f4-b286c13fb786','1ba80edb-a9cb-474d-a9e6-e513b0603c58','310de9ef-30f4-4123-ad2c-6c3e2bb8cdb8','20562b24-0576-4fc7-b017-69f3f3ccc63b','798f6ac9-f091-40c9-989f-56db13ad6a47','6ec9516c-85ea-45e9-8ab4-0093f3a91e2f','9df7552a-31cf-485e-921b-df523f724704','ec138bc5-e3eb-4cf4-87d2-e7579a9f6251','af8cb284-e6c3-47ca-b8b1-40c443f57341','64a642ba-e69e-4880-922c-edf34f504555','171efce3-6c24-4374-80ff-f06938082a4f','ceb2b419-1ef8-41f7-bb11-9d18df5d57c7','b8697e03-5a59-4bf1-aad7-541e0428d259','362a533c-6a8a-4b17-bc3f-ff9cfc142db3','82f7ee3c-0c78-4ac5-9a90-504c6e1c5f61','a3088f2d-b3a0-45c0-8664-b7c71dc4cd0b','a5de082b-ecad-4b6b-ad31-be924d507c77','7598d421-a0de-4f2f-ae81-e6ad1d58678f','24ec6dbf-6a7a-43fe-bde7-da8e87280e0f','46d535a0-a696-47b9-b3fb-1c245866e275','66d80951-c89d-4662-a7c8-904a0ad9de4f','74d4644c-6531-47cd-8e38-a372987bc87e','9b85a97d-7784-4d81-93b2-842cfc9a913f','1ab7e146-7e4b-4998-b71a-3d7a9edc6f17','f0c364af-fa8a-4c8d-8510-3d1ad58b3dee','3edcede7-5fb6-40ae-bb74-45748a2f8b04','ebbfa0b3-96d6-436f-83eb-7df4fa5f1753','31c0be34-4583-4914-bbf5-fd00b1eff51f','37146b77-3cf6-41e0-9f22-ebc5150e8b55','3c486663-aff8-471a-816b-32755038f8f1','27b815e5-a0ce-4c30-bd2b-26d85581817d','f7166b7a-6973-4b39-a16b-b8fbe3fe9cc1','feea72b2-2773-43a7-99af-916ac0b76199','eccd43b9-5fe5-4f61-9037-958e696fe794','89d86823-deea-4f9f-8fa8-aeb5a954e9e2','c116d586-a9df-4d63-a2b5-7e5c433d34c9','867b7238-5ae5-4938-a9cd-68a740cc4e21','b9c6a7e6-8024-4711-afbe-1f7024b054c4','08ff8eb0-eef2-4cd6-ad6e-24cfede8dc88','0c7c8510-5563-4676-8959-769a06cacb80','3ed829cf-810e-453b-9dcb-e522b81344b9','4759b5fd-55fa-4029-8b2b-8ea57498efe7','3a2cf3e9-867c-4245-aa08-7da53a1cddf0','05aae4f7-de30-4e26-96a9-a4f1229cc9ba','498ef53f-2fe5-4b37-8cce-a347fe2f7864','193065b8-1e38-4271-8a34-6162173ab439','e87822bd-65e9-475a-aab3-039336777ec6','a8177ff6-52df-4029-aaff-fb67f98b7c63','3f2bc1d0-9331-4d92-9e4d-7c4cdc2c3d27','22121808-fc8f-4e33-a24d-5cc22ca05efa','4faa7336-d281-484e-ae56-18def0883cac','e204e675-27e4-448f-99f0-12aa4c9f43d1','ac3856d2-afc3-4a11-b9ee-a103cba9d318','54bf5ada-91b3-4715-b3d7-7280f1698d9e','f868dc83-b00a-4e3b-ac80-5cbf1894bbd4','8bb4a648-1d86-4380-970a-d73ab9d8a0e2','bff3fa35-78e8-46f9-af03-f4eb9ffe08c5','88948313-4a10-4073-847e-eeca1014f4fd','07021bee-bc6c-4722-8770-202430afa4ff','29edcd57-f9a1-48b4-a543-d113eaf6794e','9f9f5584-5b25-413c-aaa9-bdc9a63feda1'}}),'97345',struct('BlockId','e0f8d838-16b6-419d-bd34-87d4e2e4bbee','SignalIds',{{'bd79ff19-7d83-4483-bee1-28b1bd8e11f7'}})}  OrderedModelArguments=off  Creator=GW00133806  LastModifiedBy=Cheng
settings OptimizationCC: BlockReduction=off  ConditionallyExecuteInputs=off  DefaultParameterBehavior=Inlined  OptimizeBlockIOStorage=off  BufferReuse=off  EnhancedBackFolding=on  OptimizeBlockOrder=speed  DifferentSizesBufferReuse=on
settings DebuggingCC: UnderspecifiedInitializationDetection=Classic  MergeDetectMultiDrivingBlocksExec=none  TasksWithSamePriorityMsg=none  ParameterTunabilityLossMsg=error
settings HardwareCC: ProdBitPerPointer=32  ProdBitPerSizeT=32  ProdBitPerPtrDiffT=32  ProdLargestAtomicInteger=Integer  ProdWordSize=32  ProdHWDeviceType=Custom Processor->Custom
settings ModelReferenceCC: EnableParallelModelReferenceBuilds=on  ParallelModelReferenceMATLABWorkerInit=Copy Base Workspace  ModelReferenceNumInstancesAllowed=Single  PropagateSignalLabelsOutOfModel=off
settings SFSimCC: SimParseCustomCode=off  MATLABDynamicMemAlloc=off
settings SFSimCC: SimUserIncludeDirs=|
  | .\McuEQ4Parse\src
  | .\RoadFusion_L3\src
settings RTWCC: Description=dSPACE Run-Time Target (for VEOS on Windows and ConfigurationDesk)  SystemTargetFile=dsrt.tlc  GenCodeOnly=on  MakeCommand=make_dsrt  TemplateMakefile=dsrt_default_tmf  RTWVerbose=off
settings RTWCC: CustomInclude=|
  | .\McuEQ4Parse\src
  | .\RoadFusion_L3\src
settings CodeAppCC: ForceParamTrailComments=on  MaxIdLength=128  OperatorAnnotations=on
settings STFCustomTargetCC: TargetLangStandard=C99 (ISO)  ParMdlRefBuildCompliant=on  ConcurrentExecutionCompliant=off  CPPClassGenCompliant=off  GRTInterface=off  SystemTargetFile=dsrt.tlc
settings GRTTargetCC: CompOptLevelCompliant=off  ConcurrentExecutionCompliant=off  CombineOutputUpdateFcns=off  MatFileLogging=off  CPPClassGenCompliant=off  UseToolchainInfoCompliant=off

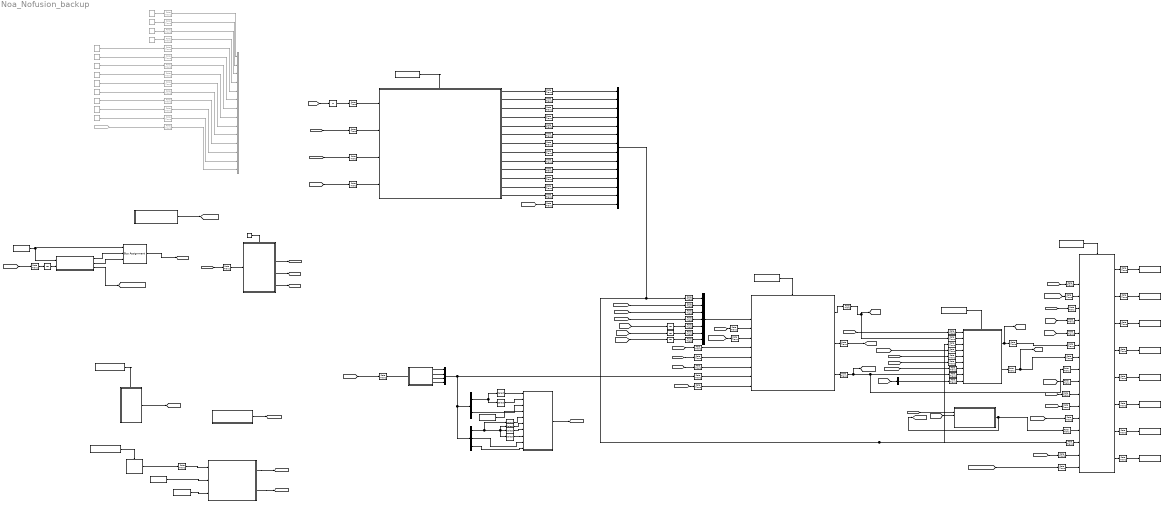
== system Noa_Nofusion_backup ==
  note: UDPReceive
  ACC_FD1 : dsmpblib/Data Outport  Priority=-10000
      settings: SourceProductName=dSPACE Model Interface Blockset
  ACC_FD2 : dsmpblib/Data Outport  Priority=-10000
      settings: SourceProductName=dSPACE Model Interface Blockset
  ACC_FD4 : dsmpblib/Data Outport  Priority=-10000
      settings: SourceProductName=dSPACE Model Interface Blockset
  Bus Assignment : BusAssignment  AssignedSignals=CSA_NODE.CSA1_MSG.LTurnLmpSwtSts,CSA_NODE.CSA1_MSG.RTurnLmpSwtSts
  Bus Creator : BusCreator  Inputs=7
  Bus Creator1 : BusCreator  Inputs=4
  Bus Creator2 : BusCreator  Commented=on  Inputs=14
  Bus Creator3 : BusCreator  Inputs=14
  Bus Selector : BusSelector  OutputSignals=EQ4_LH.EQ4_LH_ELEM,EQ4_LH.EQ4_LH_HDR
  Bus Selector1 : BusSelector  OutputSignals=LSM_HWA.RoadWidth
  Bus Selector2 : BusSelector  OutputSignals=EQ4_LA.EQ4_LA_ELEM,EQ4_LA.EQ4_LA_HDR,EQ4_LRE.EQ4_LRE_ELEM
  CAL : Subsystem
  CR_RSDS_Input : Subsystem
  CSA_Pack : Subsystem
  Chassis1 : Subsystem
  Common : Subsystem  Tag=<DSModel=3_'Fusion'>
      settings: AttributesFormatString=<DSModel='Fusion'>
  Constant : Constant  Commented=on  Value=0  OutDataTypeStr=Bus: TOS_ACCP0_BUS
  Constant1 : Constant  Commented=on  Value=0  OutDataTypeStr=Bus: TOS_ACCP1_BUS
  Constant10 : Constant  Commented=on  Value=0  OutDataTypeStr=Bus: TOS_AEB_JAOBJ_BUS
  Constant11 : Constant  Commented=on  Value=0  OutDataTypeStr=Bus: TOS_P0_TARGET_LINE_BUS
  Constant12 : Constant  Commented=on  Value=0  OutDataTypeStr=uint32
  Constant2 : Constant  Commented=on  Value=0  OutDataTypeStr=Bus: TOS_ACCP2_BUS
  Constant3 : Constant  Commented=on  Value=0  OutDataTypeStr=Bus: TOS_ACCP3_BUS
  Constant4 : Constant  Commented=on  Value=0  OutDataTypeStr=Bus: TOS_ACCP4_BUS
  Constant5 : Constant  Commented=on  Value=0  OutDataTypeStr=Bus: TOS_ACCP5_BUS
  Constant6 : Constant  Commented=on  Value=0  OutDataTypeStr=Bus: TOS_ELK_BUS
  Constant7 : Constant  Commented=on  Value=0  OutDataTypeStr=Bus: TOS_LCKIE_BUS
  Constant8 : Constant  Commented=on  Value=0  OutDataTypeStr=Bus: TOS_AEB_LONOBJ_BUS
  Constant9 : Constant  Commented=on  Value=0  OutDataTypeStr=Bus: TOS_AEB_LATOBJ_BUS
  Control1 : Subsystem
  EQ4_Lane_Pack1 : Subsystem
  From12 : From  Commented=on  GotoTag=LC_Obj
  Function-Call Generator3 : simulink/Ports & Subsystems/Function-Call Generator  sample_time=0.02  numberOfIterations=1  DisallowWideOutput=off
  IFC_FD{1..3,5..6} (5 alike) : dsmpblib/Data Outport  Priority=-10000
      settings: SourceProductName=dSPACE Model Interface Blockset
  IfRFM_LANES_In : dsmpblib/Data Inport  Priority=10000
      settings: SourceProductName=dSPACE Model Interface Blockset
  LPV : Subsystem
  RFM_Road : dsmpblib/Data Inport  Priority=10000
      settings: SourceProductName=dSPACE Model Interface Blockset
  Rate Transition{1..46,61..88} (74 alike) : RateTransition  Integrity=off  Deterministic=off
  Rate Transition{47..60} (14 alike) : RateTransition  Commented=on  Integrity=off  Deterministic=off
  Selector1 : Selector  InputPortWidth=4  IndexOptions=Index vector (dialog)  Indices=1  OutputSizes=1
  Selector2 : Selector  InputPortWidth=4  IndexOptions=Index vector (dialog)  Indices=2  OutputSizes=1
  Selector3 : Selector  InputPortWidth=4  IndexOptions=Index vector (dialog)  Indices=3  OutputSizes=1
  Selector4 : Selector  InputPortWidth=2  IndexOptions=Index vector (dialog)  Indices=1  OutputSizes=1
  Selector5 : Selector  InputPortWidth=2  IndexOptions=Index vector (dialog)  Indices=2  OutputSizes=1
  Selector6 : Selector  InputPortWidth=4  IndexOptions=Index vector (dialog)  Indices=4  OutputSizes=1
  Software-Triggered Runnable Function{,1..3} (4 alike) : dsmpblib/Software-Triggered Runnable Function
      settings: SourceProductName=dSPACE Model Interface Blockset
  Subsystem1 : Subsystem
  Subsystem2 : Subsystem
  Subsystem3 : Subsystem
  Subsystem4 : Subsystem
  UDP Receive (3)\Data Received : dsmpblib/Hardware-Triggered Runnable Function
      settings: SourceProductName=dSPACE Model Interface Blockset
  UDP Receive 2\Data Received : dsmpblib/Hardware-Triggered Runnable Function
      settings: SourceProductName=dSPACE Model Interface Blockset
  UDP_Received : Subsystem
  Unit Delay{,1..4} (5 alike) : UnitDelay  SampleTime=-1  HasFrameUpgradeWarning=on
  VCANBus : dsmpblib/Data Inport  Priority=10000
      settings: SourceProductName=dSPACE Model Interface Blockset
  aeb : Subsystem  Tag=<DSModel=2_'Osm'>
      settings: AttributesFormatString=<DSModel='Osm'>
  ifLaneBus_out_In : dsmpblib/Data Inport  Priority=10000
      settings: SourceProductName=dSPACE Model Interface Blockset
  wires:
  [RoadBus] -> Rate Transition14/1  "roadbus"
  [RoadBus] -> Rate Transition38/1
  [IfCANBus] -> Rate Transition19/1
  [LATBus] -> Unit Delay1/1
  [IfVIEBus] -> aeb/2(IfVIEBus)
  Unit Delay3/1 -> Rate Transition39/1  "aebbus"
  Control1/1(IfLONBus) -> [LONBus], Rate Transition87/1
  [AEBBus] -> Unit Delay3/1
  Rate Transition18/1 -> Bus Creator/5  "lonbus"
  [IfEHRBus] -> Rate Transition36/1
  Control1/2(IfLATBus) -> Rate Transition88/1
  [IfVIEBus] -> Rate Transition37/1
  [IfLineBus] -> Rate Transition35/1
  [LONBus] -> Unit Delay2/1
  aeb/1(IfAEBSBus) -> Rate Transition43/1, [AEBBus]
  Rate Transition20/1 -> Bus Creator/6  "latbus"
  [visMsg] -> Rate Transition16/1
  ifLaneBus_out_In/1 -> Subsystem4/4(lanebus)  "lanebus"
  [IfLineBus] -> Rate Transition13/1  "lanebus"
  [ifObjectBus] -> Rate Transition12/1
  [ifVSMBus] -> aeb/3(IfVSMBus)
  UDP Receive 2\Data Received/1 -> UDP_Received/Trigger
  UDP_Received/1(visMsg) -> [visMsg]
  Rate Transition16/1 -> Chassis1/11(IfVEQ4Bus)
  EQ4_Lane_Pack1/2(EQ4_LA) -> Bus Creator1/2  "EQ4_LA"
  EQ4_Lane_Pack1/3(EQ4_LH) -> Bus Creator1/3  "EQ4_LH"
  EQ4_Lane_Pack1/4(EQ4_LRE) -> Bus Creator1/4  "EQ4_LRE"
  Bus Creator/1 -> LPV/3(IfALLBus)
  Rate Transition22/1 -> LPV/4(IfCANBus)
  Rate Transition23/1 -> LPV/6(IfDMSBus)
  [IfCANBus] -> Rate Transition22/1
  Rate Transition29/1 -> LPV/7(IfEHRBus)
  [IfDMSBus] -> Rate Transition23/1
  Rate Transition30/1 -> LPV/8(IfVIEBus)
  [IfVIEBus] -> Rate Transition30/1
  [IfEHRBus] -> Rate Transition29/1
  Rate Transition31/1 -> EQ4_Lane_Pack1/1(In1)  "visMsg"
  Rate Transition32/1 -> LPV/9(IfEQ4Bus)
  Rate Transition19/1 -> Control1/1(IfVCANBus)
  Rate Transition33/1 -> Control1/2(IfVSMBus)
  Rate Transition34/1 -> Control1/3(IfTOSBus)
  Rate Transition35/1 -> Control1/4(IfRFMBus)
  Rate Transition36/1 -> Control1/5(IfEHRBus)
  Rate Transition37/1 -> Control1/6(IfVIEBus)
  Rate Transition38/1 -> Control1/7(IfRoadBus)
  [visMsg] -> Rate Transition31/1
  LPV/2(IfLSMBus) -> Rate Transition85/1
  Rate Transition10/1 -> Bus Creator/1
  Rate Transition12/1 -> Bus Creator/2
  Rate Transition13/1 -> Bus Creator/3  "lanebus"
  Rate Transition14/1 -> Bus Creator/4  "roadbus"
  Unit Delay2/1 -> Rate Transition18/1  "lonbus"
  Unit Delay1/1 -> Rate Transition20/1  "latbus"
  Rate Transition39/1 -> Bus Creator/7  "aebbus"
  [IfLineBus] -> Rate Transition1/1  "lanebus"
  Rate Transition1/1 -> Chassis1/14(LaneBus)  "lanebus"
  [IfCANBus] -> Rate Transition42/1
  CAL/1(IfCALBus) -> [IfCALBus]
  [IfCALBus] -> Rate Transition5/1
  Rate Transition5/1 -> LPV/5(IfCALBus)
  [IfCALBus] -> Rate Transition41/1
  [IfVIEBus] -> Rate Transition40/1
  [IfLSMBus] -> Rate Transition17/1
  [IfEHRBus] -> Rate Transition6/1
  [IfDMSBus] -> Rate Transition4/1
  Rate Transition6/1 -> Chassis1/12(IfEHRBus)
  Rate Transition4/1 -> Chassis1/13(IfDMSBus)
  [RoadBus] -> Rate Transition45/1  "roadbus"
  [ifVSMBus] -> Rate Transition26/1
  Rate Transition7/1 -> Chassis1/9(IfLatCtrlBus)
  Rate Transition8/1 -> Chassis1/8(IfLonCtrlBus)
  Rate Transition17/1 -> Chassis1/7(IfLSMBus)
  Rate Transition26/1 -> Chassis1/6(IfVSMBus)
  Rate Transition40/1 -> Chassis1/5(IfVIEBus)
  Rate Transition41/1 -> Chassis1/4(IfCALBus)
  Rate Transition42/1 -> Chassis1/3(IfVCANBus)
  Rate Transition43/1 -> Chassis1/15(IfAEBBus)  "lanebus"
  Rate Transition44/1 -> Chassis1/16(IfOSMBus)  "lanebus"
  Rate Transition45/1 -> Chassis1/17(RoadBus)  "lanebus"
  Function-Call Generator3/1 -> Common/Trigger
  [IfCANBus] -> Rate Transition3/1
  Common/2(IfDMSBus) -> [IfDMSBus]
  Common/4(IfEHRBus) -> [IfEHRBus]
  Common/3(IfVIEBus) -> [IfVIEBus]
  Rate Transition3/1 -> Common/1(IfCANBus)  "lonbus"
  LPV/3(IfPlanbus) -> Rate Transition86/1
  Rate Transition9/1 -> Control1/8(IfPlanbus)
  [RFM_LANES] -> Rate Transition11/1
  Rate Transition11/1 -> LPV/10(RFM_LANES)
  EQ4_Lane_Pack1/1(EQ4_LAP) -> Bus Creator1/1  "EQ4_LAP"
  Chassis1/8(ACC_FD4) -> Rate Transition83/1
  Chassis1/2(IFC_FD2) -> Rate Transition27/1
  Chassis1/3(IFC_FD3) -> Rate Transition46/1
  Chassis1/4(IFC_FD5) -> Rate Transition79/1
  Chassis1/5(IFC_FD6) -> Rate Transition80/1
  Chassis1/6(ACC_FD1) -> Rate Transition81/1
  Chassis1/7(ACC_FD2) -> Rate Transition82/1
  Rate Transition15/1 -> Chassis1/10(IfPlanbus)
  Rate Transition21/1 -> Subsystem1/1(l3_RFMResult)  "lonbus"
  IfRFM_LANES_In/1 -> Subsystem1/3(lane)
  RFM_Road/1 -> Subsystem1/2(RFM_Road)
  Subsystem1/1(IfRFM_LANES_In) -> [RFM_LANES]
  Subsystem1/2(roadbus) -> [RoadBus]  "roadbus"
  Subsystem3/1(Out2) -> Rate Transition21/1
  UDP Receive (3)\Data Received/1 -> Subsystem3/Trigger
  CR_RSDS_Input/1(LC_Obj) -> [LC_Obj]
  Selector4/1 -> Subsystem4/1(EQ4_LH_ELEM_0)
  Selector5/1 -> Subsystem4/2(EQ4_LH_ELEM_1)
  Bus Selector/1 -> Selector4/1, Selector5/1  "<EQ4_LH_ELEM>"
  Bus Selector/2 -> Subsystem4/3(LH_HDR)  "<EQ4_LH_HDR>"
  Subsystem4/1(Out1) -> [IfLineBus]
  [IfLSMBus] -> Bus Selector1/1
  Rate Transition24/1 -> Control1/9(roadwidth)
  Bus Selector1/1 -> Rate Transition24/1  "<RoadWidth>"
  Selector6/1 -> Subsystem4/8(EQ4_LA_ELEM_3)
  Selector3/1 -> Subsystem4/7(EQ4_LA_ELEM_2)
  Bus Selector2/3 -> Subsystem4/10(In10)  "<EQ4_LRE_ELEM>"
  Bus Selector2/1 -> Selector1/1, Selector2/1, Selector6/1, Selector3/1  "<EQ4_LA_ELEM>"
  Bus Selector2/2 -> Subsystem4/9(LA_HDR)  "<EQ4_LA_HDR>"
  Selector2/1 -> Subsystem4/6(EQ4_LA_ELEM_1)
  Bus Creator1/1 -> Bus Selector2/1, Bus Selector/1, Rate Transition32/1
  Selector1/1 -> Subsystem4/5(EQ4_LA_ELEM_0)
  Chassis1/1(IFC_FD1) -> Rate Transition25/1
  CSA_Pack/1(LTurnLmpSwtSts) -> Bus Assignment/2
  [ifPlanbus] -> Rate Transition2/1
  Unit Delay4/1 -> CSA_Pack/2(PLAN_ALC_DECS)
  Rate Transition2/1 -> Unit Delay4/1
  CSA_Pack/3(CSASim_IDC_L2_LampReq) -> [CSASim_IDC_L2_LampReq]
  [CSASim_IDC_L2_LampReq] -> Rate Transition28/1
  Rate Transition28/1 -> Chassis1/18(CSASim_IDC_L2_LampReq)
  VCANBus/1 -> CSA_Pack/1(VCAN), Bus Assignment/1
  Constant7/1 -> Rate Transition52/1
  Constant9/1 -> Rate Transition54/1
  Constant/1 -> Rate Transition58/1  "TOS_ACCP0"
  Constant1/1 -> Rate Transition59/1
  Constant3/1 -> Rate Transition48/1
  Rate Transition52/1 -> Bus Creator2/8  "TOS_LCKIE"
  Rate Transition50/1 -> Bus Creator2/6  "TOS_ACCP5"
  Rate Transition54/1 -> Bus Creator2/10  "TOS_AEB_LATOBJ"
  Rate Transition57/1 -> Bus Creator2/12  "TOS_P0_TARGET_LINE"
  Constant5/1 -> Rate Transition50/1
  Rate Transition55/1 -> Bus Creator2/11  "TOS_AEB_JAOBJ"
  Rate Transition53/1 -> Bus Creator2/9  "TOS_AEB_LONOBJ"
  Rate Transition56/1 -> Bus Creator2/13  "TOS_UpdateCnt"
  Rate Transition48/1 -> Bus Creator2/4  "TOS_ACCP3"
  Rate Transition58/1 -> Bus Creator2/1  "TOS_ACCP0"
  Rate Transition51/1 -> Bus Creator2/7  "TOS_ELK"
  Rate Transition47/1 -> Bus Creator2/3  "TOS_ACCP2"
  Constant12/1 -> Rate Transition56/1
  Constant10/1 -> Rate Transition55/1
  Constant6/1 -> Rate Transition51/1
  Rate Transition49/1 -> Bus Creator2/5  "TOS_ACCP4"
  Constant8/1 -> Rate Transition53/1
  Constant11/1 -> Rate Transition57/1
  Rate Transition59/1 -> Bus Creator2/2  "TOS_ACCP1"
  Constant2/1 -> Rate Transition47/1
  Constant4/1 -> Rate Transition49/1
  From12/1 -> Rate Transition60/1  "TOS_LC"
  Rate Transition60/1 -> Bus Creator2/14  "TOS_LC"
  [ifVSMBus] -> Unit Delay/1
  Rate Transition74/1 -> Bus Creator3/14  "TOS_LC"
  Bus Creator3/1 -> Rate Transition44/1, Rate Transition34/1, Rate Transition10/1  "IfTOSBus"
  Rate Transition76/1 -> Bus Creator3/1  "TOS_ACCP0"
  Unit Delay/1 -> Rate Transition78/1
  [IfVIEBus] -> Rate Transition67/1
  [IfCANBus] -> Rate Transition73/1
  Rate Transition78/1 -> Subsystem2/1(IfStateMBus)
  Rate Transition67/1 -> Subsystem2/2(IfVIEBus)
  Rate Transition73/1 -> Subsystem2/3(IfVCAN)
  Rate Transition75/1 -> Bus Creator3/12  "TOS_P0_TARGET_LINE"
  Rate Transition77/1 -> Bus Creator3/2  "TOS_ACCP1"
  Rate Transition62/1 -> Bus Creator3/3  "TOS_ACCP2"
  Rate Transition63/1 -> Bus Creator3/4  "TOS_ACCP3"
  Rate Transition64/1 -> Bus Creator3/5  "TOS_ACCP4"
  Rate Transition65/1 -> Bus Creator3/6  "TOS_ACCP5"
  Rate Transition66/1 -> Bus Creator3/7  "TOS_ELK"
  Rate Transition68/1 -> Bus Creator3/8  "TOS_LCKIE"
  [LC_Obj] -> Rate Transition74/1  "TOS_LC"
  Rate Transition69/1 -> Bus Creator3/9  "TOS_AEB_LONOBJ"
  Rate Transition70/1 -> Bus Creator3/10  "TOS_AEB_LATOBJ"
  Rate Transition71/1 -> Bus Creator3/11  "TOS_AEB_JAOBJ"
  Rate Transition72/1 -> Bus Creator3/13  "TOS_UpdateCnt"
  Subsystem2/1(TOS_ACCP0) -> Rate Transition76/1  "TOS_ACCP0"
  Subsystem2/2(TOS_ACCP1) -> Rate Transition77/1
  Subsystem2/3(ACCP2) -> Rate Transition62/1
  Subsystem2/4(ACCP3) -> Rate Transition63/1
  Subsystem2/5(TOS_ACCP4) -> Rate Transition64/1
  Subsystem2/6(TOS_ACCP5) -> Rate Transition65/1
  Subsystem2/7(TOS_ELK) -> Rate Transition66/1
  Subsystem2/8(TOS_LCKIE) -> Rate Transition68/1
  Subsystem2/9(TOS_AEB_LONOBJ) -> Rate Transition69/1
  Subsystem2/10(TOS_AEB_LATOBJ) -> Rate Transition70/1
  Subsystem2/11(TOS_AEB_JAOBJ) -> Rate Transition71/1
  Subsystem2/12(TOS_P0_TARGET_LINE) -> Rate Transition75/1
  Subsystem2/13(TOS_UpdateCnt) -> Rate Transition72/1
  [visMsg] -> Rate Transition61/1
  Rate Transition61/1 -> Subsystem2/4(visMsg)
  Software-Triggered Runnable Function/1 -> Subsystem2/Trigger
  Bus Assignment/1 -> [IfCANBus]
  CSA_Pack/2(RTurnLmpSwtSts) -> Bus Assignment/3
  Software-Triggered Runnable Function1/1 -> LPV/Trigger
  Software-Triggered Runnable Function2/1 -> Control1/Trigger
  Software-Triggered Runnable Function3/1 -> Chassis1/Trigger
  Rate Transition25/1 -> IFC_FD1/1
  Rate Transition27/1 -> IFC_FD2/1
  Rate Transition46/1 -> IFC_FD3/1
  Rate Transition79/1 -> IFC_FD5/1
  Rate Transition80/1 -> IFC_FD6/1
  Rate Transition81/1 -> ACC_FD1/1
  Rate Transition82/1 -> ACC_FD2/1
  Rate Transition83/1 -> ACC_FD4/1
  Rate Transition84/1 -> [ifVSMBus], Rate Transition33/1  "VSM_CTRL_LINE"
  LPV/1(IfVSMBus) -> Rate Transition84/1  "VSM_CTRL_LINE"
  Rate Transition86/1 -> Rate Transition9/1, Rate Transition15/1, [ifPlanbus]  "VSM_CTRL_LINE"
  Rate Transition85/1 -> [IfLSMBus]  "VSM_CTRL_LINE"
  Rate Transition87/1 -> Rate Transition8/1
  Rate Transition88/1 -> Rate Transition7/1, [LATBus]
